simulink model "PID_Controller"  (R2017b)
settings: Solver=VariableStepAuto  StartTime=0.0  StopTime=10.0  RelTol=1e-3  EnableMultiTasking=on
values from neighbouring files (symbols this model uses):
  Fmatrix = [-1/sqrt(2) 0 1/sqrt(2) 1 ... (first row only)    [I_F_matrices.m]
  Imatrix = [1 0 0 1/2 ... (first row only)    [I_F_matrices.m]
libraries: dspmtrx3 x1, dspinverses x1
(part 2 of 5)

== matlab function PID_Controller/tau/Centrifugal and Coriolis Matrix/C_matrix ==
  data: in1 input; C output; in2 input
function C = Cmatrix(in1,in2)

C=zeros(6,6);
%CMATRIX
%    C = CMATRIX(IN1,IN2)

%    This function was generated by the Symbolic Math Toolbox version 7.0.
%    08-Aug-2017 18:04:25

dq1 = in2(1,:);
dq2 = in2(2,:);
dq3 = in2(3,:);
dq4 = in2(4,:);
dq5 = in2(5,:);
dq6 = in2(6,:);
q1 = in1(1,:);
q2 = in1(2,:);
q3 = in1(3,:);
q4 = in1(4,:);
q5 = in1(5,:);
q6 = in1(6,:);
t2 = cos(q1);
t3 = cos(q2);
t4 = sin(q1);
t5 = sin(q3);
t6 = cos(q3);
t7 = sin(q2);
t8 = t2.*(1.0./4.0);
t9 = t3.*t4.*(1.0./2.0);
t10 = t8+t9;
t11 = t4.*(1.0./4.0);
t19 = t2.*t3.*(1.0./2.0);
t12 = t11-t19;
t13 = t2.*t3.*t5;
t14 = t2.*t6.*t7;
t15 = t13+t14;
t16 = t3.*t4.*t5;
t17 = t4.*t6.*t7;
t18 = t16+t17;
t20 = t2.*t3.*t6;
t23 = t2.*t5.*t7;
t21 = t20-t23;
t22 = t3.*t4.*t6;
t24 = t3.*t6;
t26 = t5.*t7;
t25 = t24-t26;
t27 = t3.*t5;
t28 = t6.*t7;
t29 = t27+t28;
t30 = sin(q5);
t31 = sin(q4);
t32 = cos(q4);
t33 = cos(q5);
t34 = t8+t9+t16+t17;
t38 = t4.*t5.*t7;
t35 = t22-t38;
t36 = -t11+t13+t14+t19;
t37 = t2.*t31;
t39 = t18.*t33;
t40 = t4.*t31;
t44 = t21.*t32;
t41 = t40-t44;
t42 = t15.*t33;
t45 = t30.*t41;
t43 = t42-t45;
t46 = t32.*(t22-t38);
t47 = t37+t46;
t48 = t30.*t47;
t49 = t39+t48;
t50 = t21.*t33;
t58 = t15.*t30.*t32;
t51 = t50-t58;
t52 = t33.*t35;
t69 = t18.*t30.*t32;
t53 = t52-t69;
t54 = t2.*t7.*(1.0./2.0);
t55 = -t20+t23+t54;
t56 = t4.*t7.*(1.0./2.0);
t57 = -t22+t38+t56;
t59 = t7.*(1.0./2.0);
t60 = -t24+t26+t59;
t61 = t25.*t33;
t63 = t29.*t30.*t32;
t62 = t61-t63;
t64 = t3.*(1.0./2.0);
t65 = t27+t28+t64;
t66 = t29.*t33;
t67 = t25.*t30.*t32;
t68 = t66+t67;
t70 = t2.*t3.*(3.0./2.0e2);
t71 = t4.*t7.*(3.0./2.0e2);
t72 = t70+t71;
t73 = t2.*t3.*(7.0./2.0e2);
t74 = t4.*t7.*(7.0./2.0e2);
t75 = t73+t74;
t76 = t3.*t4.*(3.0./2.0e2);
t77 = t3.*t4.*(7.0./2.0e2);
t147 = t2.*t7.*(7.0./2.0e2);
t78 = t77-t147;
t79 = t34.*t43.*(1.0./2.0);
t80 = t34.*t51;
t81 = t34.*t43;
t82 = t34.*t51.*(1.0./2.0);
t166 = t36.*t49;
t83 = t81-t166;
t84 = t7.*t21.*(1.0./2.0);
t85 = t12.*t29;
t86 = t7.*t15.*(8.0./5.0);
t226 = t12.*t25.*(1.6e1./5.0);
t87 = t86-t226;
t88 = t7.*t15.*(1.0./2.0);
t230 = t12.*t25;
t89 = t88-t230;
t90 = t7.*t21.*(8.0./5.0);
t91 = t12.*t29.*(1.6e1./5.0);
t92 = t49.*t60.*(1.0./2.0);
t93 = t34.*t62.*(1.0./2.0);
t94 = t92+t93;
t95 = t34.*t68;
t96 = t49.*t60;
t97 = t34.*t62;
t98 = t96+t97;
t99 = t34.*t68.*(1.0./2.0);
t100 = t43.*t60.*(1.0./2.0);
t101 = t36.*t62.*(1.0./2.0);
t102 = t36.*t68;
t103 = t100+t101;
t104 = t43.*t60;
t105 = t36.*t62;
t106 = t36.*t68.*(1.0./2.0);
t107 = t104+t105;
t108 = t10.*t15;
t109 = t12.*t18;
t110 = t108+t109;
t111 = t10.*t21.*(1.6e1./5.0);
t112 = t12.*t35.*(1.6e1./5.0);
t113 = t10.*t21;
t114 = t10.*t15.*(1.6e1./5.0);
t115 = t12.*t18.*(1.6e1./5.0);
t116 = t114+t115;
t117 = t12.*t35;
t118 = t7.*t35.*(1.0./2.0);
t119 = t10.*t25.*(1.6e1./5.0);
t120 = t7.*t18.*(8.0./5.0);
t121 = t119+t120;
t122 = t10.*t25;
t123 = t7.*t18.*(1.0./2.0);
t124 = t122+t123;
t125 = t7.*t35.*(8.0./5.0);
t126 = t2.*t31.*(1.0./2.0e2);
t150 = t4.*t32.*(1.0./2.0e2);
t127 = t126-t150;
t128 = t2.*t32.*(3.0./1.0e3);
t129 = t4.*t31.*(3.0./1.0e3);
t130 = t128+t129;
t131 = t2.*t31.*(3.0./1.0e3);
t153 = t4.*t32.*(3.0./1.0e3);
t132 = t131-t153;
t133 = t2.*t32.*(1.0./2.0e2);
t134 = t4.*t31.*(1.0./2.0e2);
t135 = t133+t134;
t136 = t15.*t31.*(1.0./2.0e2);
t404 = t18.*t32.*(1.0./2.0e2);
t137 = t136-t404;
t138 = t15.*t32.*(3.0./1.0e3);
t139 = t18.*t31.*(3.0./1.0e3);
t140 = t138+t139;
t141 = t15.*t31.*(3.0./1.0e3);
t399 = t18.*t32.*(3.0./1.0e3);
t142 = t141-t399;
t143 = t15.*t32.*(1.0./2.0e2);
t144 = t18.*t31.*(1.0./2.0e2);
t145 = t143+t144;
t157 = t2.*t7.*(3.0./2.0e2);
t146 = t76-t157;
t148 = t3.*t78;
t149 = t7.*t72;
t151 = t32.*t127;
t179 = t31.*t130;
t152 = t151-t179;
t154 = t32.*t132;
t182 = t31.*t135;
t155 = t154-t182;
t156 = t3.*t72;
t158 = t7.*t146;
t159 = t32.*t135;
t160 = t31.*t132;
t161 = t159+t160;
t162 = t32.*t130;
t163 = t31.*t127;
t164 = t162+t163;
t194 = t36.*t49.*(1.0./2.0);
t165 = t79-t194;
t167 = t33.*t41;
t168 = t15.*t30;
t169 = t167+t168;
t170 = t18.*t30;
t172 = t33.*t47;
t171 = t170-t172;
t173 = t25.*t30;
t174 = t29.*t32.*t33;
t175 = t173+t174;
t176 = t4.*t32;
t177 = t21.*t31;
t178 = t176+t177;
t180 = t2.*t32;
t183 = t31.*t35;
t181 = t180-t183;
t184 = t32.*t181.*(1.0./2.0e2);
t185 = t31.*t178.*(1.0./2.0e2);
t186 = t184+t185;
t187 = t32.*t178.*(3.0./1.0e3);
t281 = t31.*t181.*(3.0./1.0e3);
t188 = t187-t281;
t189 = t32.*t181.*(3.0./1.0e3);
t190 = t31.*t178.*(3.0./1.0e3);
t191 = t189+t190;
t192 = t32.*t178.*(1.0./2.0e2);
t276 = t31.*t181.*(1.0./2.0e2);
t193 = t192-t276;
t195 = t34.*t169;
t534 = t36.*t171;
t196 = t195-t534;
t197 = t165.*t196.*(1.0./2.0);
t198 = t34.*t169.*(1.0./2.0);
t467 = t36.*t171.*(1.0./2.0);
t199 = t198-t467;
t200 = t83.*t199.*(1.0./2.0);
t201 = cos(q6);
t202 = sin(q6);
t203 = t60.*t171.*(1.0./2.0);
t204 = t34.*t175.*(1.0./2.0);
t205 = t203+t204;
t206 = t98.*t205.*(1.0./2.0);
t207 = t60.*t171;
t208 = t34.*t175;
t209 = t207+t208;
t210 = t94.*t209.*(1.0./2.0);
t211 = t2.*t201.*(2.0./1.25e2);
t212 = t4.*t202.*(2.0./1.25e2);
t213 = t211+t212;
t214 = t2.*t202.*(2.0./1.25e2);
t316 = t4.*t201.*(2.0./1.25e2);
t215 = t214-t316;
t216 = t60.*t169;
t217 = t36.*t175;
t218 = t216+t217;
t219 = t103.*t218.*(1.0./2.0);
t220 = t60.*t169.*(1.0./2.0);
t221 = t36.*t175.*(1.0./2.0);
t222 = t220+t221;
t223 = t107.*t222.*(1.0./2.0);
t224 = t2.*t7.*t18.*(1.0./2.0);
t225 = t2.*t7.*t18.*(8.0./5.0);
t227 = t3.*t15.*(1.0./2.0);
t353 = t2.*t7.*t25.*(1.0./2.0);
t228 = t84+t85+t227-t353;
t229 = t87.*t228.*(1.0./2.0);
t231 = t3.*t15.*(8.0./5.0);
t274 = t2.*t7.*t25.*(8.0./5.0);
t232 = t90+t91+t231-t274;
t233 = t89.*t232.*(1.0./2.0);
t234 = t49.*t55;
t354 = t36.*t53;
t355 = t43.*t57;
t235 = t80+t234-t354-t355;
t236 = t49.*t55.*(1.0./2.0);
t302 = t36.*t53.*(1.0./2.0);
t303 = t43.*t57.*(1.0./2.0);
t237 = t82+t236-t302-t303;
t238 = t51.*t60;
t239 = t55.*t62;
t240 = t51.*t60.*(1.0./2.0);
t241 = t55.*t62.*(1.0./2.0);
t242 = t53.*t60;
t243 = t57.*t62;
t244 = t53.*t60.*(1.0./2.0);
t245 = t57.*t62.*(1.0./2.0);
t246 = t3.*t146;
t247 = t7.*t75;
t248 = t3.*t18.*(1.0./2.0);
t358 = t10.*t29;
t359 = t4.*t7.*t25.*(1.0./2.0);
t360 = t118+t248-t358-t359;
t249 = t121.*t360.*(1.0./2.0);
t250 = t3.*t18.*(8.0./5.0);
t252 = t10.*t29.*(1.6e1./5.0);
t253 = t4.*t7.*t25.*(8.0./5.0);
t254 = t125+t250-t252-t253;
t251 = t124.*t254.*(1.0./2.0);
t331 = t43.*t65.*(1.0./2.0);
t255 = t106-t240+t241-t331;
t341 = t49.*t65.*(1.0./2.0);
t256 = t99-t244+t245-t341;
t257 = t30.*t60.*t178.*(1.0./2.0);
t443 = t29.*t30.*t31.*t36.*(1.0./2.0);
t258 = t257-t443;
t259 = t107.*t258.*(1.0./2.0);
t260 = t30.*t60.*t178;
t511 = t29.*t30.*t31.*t36;
t261 = t260-t511;
t262 = t103.*t261.*(1.0./2.0);
t273 = t29.*t31.*(1.09e2./1.0e3);
t263 = t59-t273;
t264 = t4.*t32.*(1.09e2./1.0e3);
t265 = t21.*t31.*(1.09e2./1.0e3);
t266 = -t11+t19+t264+t265;
t267 = t15.*t31.*(1.09e2./1.0e3);
t268 = t54+t267;
t269 = t31.*(t22-t38).*(1.09e2./1.0e3);
t315 = t2.*t32.*(1.09e2./1.0e3);
t270 = t8+t9+t269-t315;
t271 = t12.*(t22-t38).*(1.6e1./5.0);
t352 = t4.*t7.*t15.*(8.0./5.0);
t272 = t111+t225+t271-t352;
t275 = t35.*t43;
t277 = t32.*t193;
t278 = t31.*t191;
t279 = t277+t278;
t280 = t2.*t279.*(1.0./2.0);
t282 = t32.*t188;
t283 = t31.*t186;
t284 = t282+t283;
t285 = t32.*t186;
t429 = t31.*t188;
t286 = t285-t429;
t287 = t4.*t286.*(1.0./2.0);
t288 = t32.*t191;
t430 = t31.*t193;
t289 = t288-t430;
t290 = t151-t154-t179+t182;
t291 = t29.*t49;
t292 = t21.*t62;
t293 = t29.*t43;
t294 = t30.*t60.*t181.*(1.0./2.0);
t295 = t29.*t30.*t31.*t34.*(1.0./2.0);
t296 = t294+t295;
t297 = t30.*t60.*t181;
t298 = t29.*t30.*t31.*t34;
t299 = t297+t298;
t300 = t159+t160-t162-t163;
t301 = t4.*t300.*(1.0./2.0);
t304 = t30.*t36.*t181;
t305 = t30.*t34.*t178;
t306 = t304+t305;
t307 = t165.*t306.*(1.0./2.0);
t308 = t30.*t36.*t181.*(1.0./2.0);
t309 = t30.*t34.*t178.*(1.0./2.0);
t310 = t308+t309;
t311 = t83.*t310.*(1.0./2.0);
t312 = t18.*t31.*(1.09e2./1.0e3);
t313 = t56+t312;
t529 = t25.*t31.*(1.09e2./1.0e3);
t314 = t64-t529;
t317 = t202.*t213;
t322 = t201.*t215;
t318 = t317-t322;
t319 = t201.*t213;
t320 = t202.*t215;
t321 = t319+t320;
t323 = t51.*t318.*(1.0./2.0);
t324 = t33.*t35.*(1.1e1./5.0e2);
t412 = t18.*t30.*t32.*(1.1e1./5.0e2);
t325 = -t22+t38+t56+t324-t412;
t339 = t30.*t47.*(1.1e1./5.0e2);
t340 = t18.*t33.*(1.1e1./5.0e2);
t326 = t8+t9+t16+t17-t339-t340;
t327 = t30.*t41.*(1.1e1./5.0e2);
t334 = t15.*t33.*(1.1e1./5.0e2);
t328 = -t11+t13+t14+t19+t327-t334;
t329 = t29.*t30.*t32.*(1.1e1./5.0e2);
t338 = t25.*t33.*(1.1e1./5.0e2);
t330 = -t24+t26+t59+t329-t338;
t332 = t21.*t33.*(1.1e1./5.0e2);
t413 = t15.*t30.*t32.*(1.1e1./5.0e2);
t333 = -t20+t23+t54+t332-t413;
t335 = t29.*t33.*(1.1e1./5.0e2);
t336 = t25.*t30.*t32.*(1.1e1./5.0e2);
t337 = t27+t28+t64+t335+t336;
t342 = t246+t247;
t343 = t2.*t342.*(1.0./2.0);
t344 = t2.*t152.*(1.0./2.0);
t363 = t7.*t78;
t345 = t156-t363;
t346 = t4.*t345.*(1.0./2.0);
t361 = t3.*t75;
t347 = t158-t361;
t348 = t4.*t347.*(1.0./2.0);
t349 = t4.*t164.*(1.0./2.0);
t350 = t12.*(t22-t38);
t619 = t4.*t7.*t15.*(1.0./2.0);
t351 = t113+t224+t350-t619;
t598 = t43.*t65;
t356 = t102-t238+t239-t598;
t604 = t49.*t65;
t357 = t95-t242+t243-t604;
t362 = t7.*(t76-t157);
t364 = t25.*t43;
t444 = t15.*t62;
t365 = t364-t444;
t366 = t255.*t365.*(1.0./2.0);
t367 = t25.*t49;
t431 = t18.*t62;
t368 = t367-t431;
t369 = t256.*t368.*(1.0./2.0);
t370 = t35.*t43.*(1.0./2.0);
t371 = t84+t85;
t372 = t87.*t371.*(1.0./2.0);
t373 = t90+t91;
t374 = t89.*t373.*(1.0./2.0);
t375 = t35.*t62;
t376 = -t95+t242+t291+t375;
t377 = t94.*t376.*(1.0./2.0);
t378 = t29.*t49.*(1.0./2.0);
t379 = t35.*t62.*(1.0./2.0);
t380 = -t99+t244+t378+t379;
t381 = t98.*t380.*(1.0./2.0);
t382 = -t102+t238+t292+t293;
t383 = t103.*t382.*(1.0./2.0);
t384 = t21.*t62.*(1.0./2.0);
t385 = t29.*t43.*(1.0./2.0);
t386 = -t106+t240+t384+t385;
t387 = t107.*t386.*(1.0./2.0);
t388 = t18.*t51;
t437 = t21.*t49;
t438 = t15.*t53;
t389 = t275+t388-t437-t438;
t390 = t165.*t389.*(1.0./2.0);
t391 = t62.*(t22-t38);
t447 = t25.*t53;
t448 = t18.*t68;
t392 = t291+t391-t447-t448;
t393 = t94.*t392.*(1.0./2.0);
t449 = t25.*t51;
t450 = t15.*t68;
t394 = t292+t293-t449-t450;
t395 = t18.*t43;
t432 = t15.*t49;
t396 = t395-t432;
t397 = t237.*t396.*(1.0./2.0);
t398 = t32.*t145;
t400 = t31.*t142;
t401 = t398+t400;
t402 = t2.*t401.*(1.0./2.0);
t403 = t32.*t140;
t405 = t31.*t137;
t406 = t403+t405;
t407 = t32.*t137;
t455 = t31.*t140;
t408 = t407-t455;
t409 = t4.*t408.*(1.0./2.0);
t410 = t32.*t142;
t456 = t31.*t145;
t411 = t410-t456;
t414 = t22-t38-t324+t412;
t415 = t53.*t328;
t416 = t62.*t328;
t417 = t20-t23-t332+t413;
t418 = t27+t28+t335+t336;
t419 = t51.*t330;
t420 = t62.*t326;
t421 = t49.*t330;
t422 = t420+t421;
t423 = t43.*t326;
t504 = t49.*t328;
t424 = t423-t504;
t439 = t21.*t49.*(1.0./2.0);
t425 = t82-t302+t370-t439;
t426 = t43.*t330;
t427 = t416+t426;
t428 = t53.*t330;
t433 = t15.*t263;
t434 = t25.*t266;
t435 = t433+t434;
t436 = t21.*t263;
t440 = t21.*t270;
t441 = t111+t271;
t442 = t18.*t266;
t445 = t18.*t263;
t446 = t125-t252;
t451 = t35.*t263;
t452 = t15.*t31.*t152.*(1.0./2.0);
t453 = t18.*t31.*t321.*(1.0./2.0);
t454 = t18.*t31.*t164.*(1.0./2.0);
t457 = (t22-t38).*(t42-t45);
t458 = t388-t437-t438+t457;
t459 = (t22-t38).*(t42-t45).*(1.0./2.0);
t460 = t82-t302-t439+t459;
t461 = t110.*t441.*(1.0./2.0);
t462 = t113+t350;
t463 = t116.*t462.*(1.0./2.0);
t464 = t118-t358;
t465 = t121.*t464.*(1.0./2.0);
t466 = t124.*t446.*(1.0./2.0);
t468 = t80-t354-t437+t457;
t469 = t165.*t468.*(1.0./2.0);
t470 = t83.*t460.*(1.0./2.0);
t471 = t15.*t164.*(1.0./2.0);
t472 = t21.*t152.*(1.0./2.0);
t473 = t35.*t321.*(1.0./2.0);
t474 = t18.*t155.*(1.0./2.0);
t475 = t35.*t164.*(1.0./2.0);
t476 = t103.*t394.*(1.0./2.0);
t477 = t15.*t300.*(1.0./2.0);
t478 = t25.*t30.*t181;
t507 = t18.*t29.*t30.*t31;
t479 = t478-t507;
t480 = t18.*t290.*(1.0./2.0);
t481 = t15.*t30.*t181;
t482 = t18.*t30.*t178;
t483 = t481+t482;
t484 = t29.*t266;
t485 = t15.*t25.*t31.*(1.09e2./5.0e2);
t486 = -t436+t484+t485;
t487 = t87.*t486.*(1.0./2.0);
t488 = t458.*(t79-t194).*(1.0./2.0);
t489 = t460.*(t395-t432).*(1.0./2.0);
t527 = t35.*t266;
t490 = t440-t527;
t532 = t15.*t270;
t491 = t441.*(t442-t532).*(1.0./2.0);
t492 = t25.*t30.*t178;
t493 = t15.*t29.*t30.*t31;
t494 = t492+t493;
t495 = t494.*(t100+t101).*(1.0./2.0);
t496 = t258.*(t364-t444).*(1.0./2.0);
t497 = t25.*t270;
t498 = t445+t497;
t499 = (t100+t101).*(t292+t293-t449-t450).*(1.0./2.0);
t500 = t29.*t270;
t501 = t18.*t25.*t31.*(1.09e2./5.0e2);
t502 = -t451+t500+t501;
t503 = t121.*t502.*(1.0./2.0);
t505 = t4.*t31.*(1.09e2./1.0e3);
t927 = t21.*t32.*(1.09e2./1.0e3);
t506 = t505-t927;
t508 = t2.*t31.*(1.09e2./1.0e3);
t509 = t32.*(t22-t38).*(1.09e2./1.0e3);
t510 = t508+t509;
t512 = t2.*t290.*(1.0./2.0);
t513 = t98.*t296.*(1.0./2.0);
t514 = t94.*t299.*(1.0./2.0);
t515 = t222.*t365.*(1.0./2.0);
t516 = t15.*t175;
t536 = t25.*t169;
t517 = t516-t536;
t518 = t15.*t171;
t537 = t18.*t169;
t519 = t518-t537;
t520 = t165.*t519.*(1.0./2.0);
t521 = t18.*t175;
t538 = t25.*t171;
t522 = t521-t538;
t523 = t205.*t368.*(1.0./2.0);
t524 = t30.*t178.*t318.*(1.0./2.0);
t525 = t30.*t181.*t321.*(1.0./2.0);
t526 = t18.*t268;
t528 = t164.*t178.*(1.0./2.0);
t530 = t15.*t314;
t531 = t152.*t181.*(1.0./2.0);
t533 = t18.*t314;
t535 = t53.*t321.*(1.0./2.0);
t539 = t33.*t41.*(1.1e1./5.0e2);
t540 = t15.*t30.*(1.1e1./5.0e2);
t541 = t539+t540;
t542 = t25.*t30.*(1.1e1./5.0e2);
t543 = t29.*t32.*t33.*(1.1e1./5.0e2);
t544 = t542+t543;
t545 = t18.*t30.*(1.1e1./5.0e2);
t561 = t33.*t47.*(1.1e1./5.0e2);
t546 = t545-t561;
t547 = t197+t200+t206+t210+t219+t223;
t548 = t62.*t414;
t549 = t49.*t418;
t550 = t49.*t417;
t594 = t51.*t326;
t778 = t43.*t414;
t551 = t415+t550-t594-t778;
t552 = t62.*t417;
t553 = t43.*t418;
t554 = t386.*t427.*(1.0./2.0);
t555 = t380.*t422.*(1.0./2.0);
t595 = t68.*t328;
t556 = t419+t552+t553-t595;
t557 = t103.*t556.*(1.0./2.0);
t591 = t68.*t326;
t558 = t428+t548+t549-t591;
t559 = t94.*t558.*(1.0./2.0);
t560 = t49.*t541;
t562 = t169.*t326;
t563 = t560+t562-t171.*t328-t43.*t546;
t564 = t165.*t563.*(1.0./2.0);
t565 = t169.*t318.*(1.0./2.0);
t566 = t175.*t328;
t567 = t169.*t330;
t1010 = t43.*t544;
t1011 = t62.*t541;
t568 = t566+t567-t1010-t1011;
t569 = t175.*t326;
t570 = t171.*t330;
t571 = t569+t570-t49.*t544-t62.*t546;
t572 = t94.*t571.*(1.0./2.0);
t573 = t205.*t422.*(1.0./2.0);
t574 = t199.*t424.*(1.0./2.0);
t575 = t222.*t427.*(1.0./2.0);
t576 = t30.*t62.*t181.*(1.1e1./5.0e2);
t577 = t29.*t30.*t31.*t49.*(1.1e1./5.0e2);
t578 = t576+t577-t30.*t181.*t330-t29.*t30.*t31.*t326;
t579 = t94.*t578.*(1.0./2.0);
t580 = t30.*t49.*t178.*(1.1e1./5.0e2);
t581 = t30.*t181.*t328;
t582 = t30.*t178.*t326;
t583 = t30.*t43.*t181.*(1.1e1./5.0e2);
t584 = t580+t581+t582+t583;
t585 = t165.*t584.*(1.0./2.0);
t586 = t30.*t62.*t178.*(1.1e1./5.0e2);
t587 = t29.*t30.*t31.*t328;
t982 = t30.*t178.*t330;
t983 = t29.*t30.*t31.*t43.*(1.1e1./5.0e2);
t588 = t586+t587-t982-t983;
t589 = t258.*t427.*(1.0./2.0);
t590 = t310.*t424.*(1.0./2.0);
t592 = t49.*t337;
t593 = t43.*t325;
t596 = t43.*t337;
t597 = t237.*t424.*(1.0./2.0);
t599 = t51.*t201.*(2.0./1.25e2);
t600 = t51.*t202.*(2.0./1.25e2);
t605 = t53.*t201.*(2.0./1.25e2);
t601 = t600-t605;
t602 = t53.*t202.*(2.0./1.25e2);
t603 = t599+t602;
t606 = t201.*t601;
t729 = t202.*t603;
t607 = t606-t729;
t608 = t2.*t607.*(1.0./2.0);
t609 = t202.*t601;
t610 = t201.*t603;
t611 = t609+t610;
t612 = t4.*t611.*(1.0./2.0);
t613 = t31.^2;
t614 = t18.*t613.*(1.0./2.0e2);
t615 = t15.*t31.*t32.*(1.0./2.0e2);
t616 = t614+t615;
t617 = t15.*t613.*(3.0./1.0e3);
t669 = t18.*t31.*t32.*(3.0./1.0e3);
t618 = t617-t669;
t620 = t15.*t31.*t201.*(2.0./1.25e2);
t621 = t18.*t31.*t202.*(2.0./1.25e2);
t622 = t620+t621;
t623 = t15.*t31.*t202.*(2.0./1.25e2);
t673 = t18.*t31.*t201.*(2.0./1.25e2);
t624 = t623-t673;
t625 = t148+t149;
t730 = t2.*t155.*(1.0./2.0);
t731 = t4.*t161.*(1.0./2.0);
t732 = t2.*t625.*(1.0./2.0);
t626 = t343+t344+t346+t348+t349-t730-t731-t732;
t627 = t116.*t351.*(1.0./2.0);
t628 = t110.*t272.*(1.0./2.0);
t629 = t83.*t237.*(1.0./2.0);
t630 = t3.*(t77-t147);
t631 = t149-t246-t247+t630;
t632 = t156-t361+t362-t363;
t633 = t25.*t43.*(1.0./2.0);
t662 = t15.*t62.*(1.0./2.0);
t634 = t633-t662;
t635 = t356.*t634.*(1.0./2.0);
t636 = t25.*t49.*(1.0./2.0);
t664 = t18.*t62.*(1.0./2.0);
t637 = t636-t664;
t638 = t357.*t637.*(1.0./2.0);
t639 = t15.*t161.*(1.0./2.0);
t640 = t15.*t53.*(1.0./2.0);
t641 = t18.*t152.*(1.0./2.0);
t691 = t25.*t53.*(1.0./2.0);
t692 = t18.*t68.*(1.0./2.0);
t642 = t378+t379-t691-t692;
t643 = t98.*t642.*(1.0./2.0);
t693 = t25.*t51.*(1.0./2.0);
t694 = t15.*t68.*(1.0./2.0);
t644 = t384+t385-t693-t694;
t645 = t107.*t644.*(1.0./2.0);
t646 = t18.*t43.*(1.0./2.0);
t695 = t15.*t49.*(1.0./2.0);
t647 = t646-t695;
t648 = t235.*t647.*(1.0./2.0);
t649 = t21.*t201.*(2.0./1.25e2);
t650 = t21.*t202.*(2.0./1.25e2);
t713 = t35.*t201.*(2.0./1.25e2);
t651 = t650-t713;
t652 = t21.*t32.*(1.0./2.0e2);
t653 = t21.*t31.*(3.0./1.0e3);
t717 = t32.*t35.*(3.0./1.0e3);
t654 = t653-t717;
t655 = t18.*t263.*(1.6e1./5.0);
t656 = t25.*t270.*(1.6e1./5.0);
t657 = t655+t656;
t936 = t15.*t313;
t658 = t440+t526-t527-t936;
t659 = t18.*t268.*(1.6e1./5.0);
t660 = t21.*t270.*(1.6e1./5.0);
t938 = t15.*t313.*(1.6e1./5.0);
t661 = t659+t660-t938-t35.*t266.*(1.6e1./5.0);
t663 = t255.*(t364-t444).*(1.0./2.0);
t941 = t25.*t268;
t665 = t436-t484+t530-t941;
t666 = t21.*t263.*(1.6e1./5.0);
t667 = t15.*t314.*(1.6e1./5.0);
t942 = t29.*t266.*(1.6e1./5.0);
t943 = t25.*t268.*(1.6e1./5.0);
t668 = t666+t667-t942-t943;
t670 = t31.*t616;
t867 = t32.*t618;
t671 = t670-t867;
t672 = t2.*t671.*(1.0./2.0);
t674 = t202.*t622;
t868 = t201.*t624;
t675 = t674-t868;
t676 = t2.*t675.*(1.0./2.0);
t677 = t32.*t616;
t678 = t31.*t618;
t679 = t677+t678;
t680 = t18.*t266.*(1.6e1./5.0);
t681 = t680-t15.*t270.*(1.6e1./5.0);
t682 = t351.*t681.*(1.0./2.0);
t683 = t272.*(t442-t532).*(1.0./2.0);
t684 = t201.*t622;
t685 = t202.*t624;
t686 = t684+t685;
t687 = t15.*t263.*(1.6e1./5.0);
t688 = t25.*t266.*(1.6e1./5.0);
t689 = t687+t688;
t712 = t18.*t51.*(1.0./2.0);
t690 = (t81-t166).*(t439-t459+t640-t712).*(1.0./2.0);
t696 = t237.*(t395-t432).*(1.0./2.0);
t932 = t25.*t313;
t697 = t451-t500+t533-t932;
t698 = t18.*t314.*(1.6e1./5.0);
t699 = t35.*t263.*(1.6e1./5.0);
t700 = t468.*(t79-t194).*(1.0./2.0);
t701 = t460.*(t81-t166).*(1.0./2.0);
t702 = t94.*(-t95+t242+t291+t375).*(1.0./2.0);
t703 = t98.*(-t99+t244+t378+t379).*(1.0./2.0);
t704 = t29.*(t42-t45);
t705 = -t102+t238+t292+t704;
t706 = t705.*(t100+t101).*(1.0./2.0);
t707 = t29.*(t42-t45).*(1.0./2.0);
t708 = -t106+t240+t384+t707;
t709 = t708.*(t104+t105).*(1.0./2.0);
t710 = t121.*(t118-t358).*(1.0./2.0);
t711 = t124.*(t125-t252).*(1.0./2.0);
t714 = t201.*t651;
t715 = t202.*(t22-t38).*(2.0./1.25e2);
t716 = t649+t715;
t718 = t32.*t654;
t719 = t31.*(t22-t38).*(1.0./2.0e2);
t720 = t652+t719;
t721 = t201.*t716;
t722 = t202.*t651;
t723 = t721+t722;
t724 = t4.*t723.*(1.0./2.0);
t725 = t32.*t720;
t726 = t31.*t654;
t727 = t725+t726;
t728 = t4.*t727.*(1.0./2.0);
t733 = t428-t591+t592-t62.*t325;
t734 = t94.*t733.*(1.0./2.0);
t735 = t49.*t337.*(1.0./2.0);
t736 = t53.*t330.*(1.0./2.0);
t737 = t43.*t325.*(1.0./2.0);
t738 = t53.*t328.*(1.0./2.0);
t757 = t49.*t333.*(1.0./2.0);
t758 = t51.*t326.*(1.0./2.0);
t739 = t737+t738-t757-t758;
t740 = t62.*t328.*(1.0./2.0);
t741 = t43.*t330.*(1.0./2.0);
t742 = t740+t741;
t1034 = t62.*t333;
t743 = t419-t595+t596-t1034;
t744 = t103.*t743.*(1.0./2.0);
t745 = t43.*t337.*(1.0./2.0);
t746 = t51.*t330.*(1.0./2.0);
t747 = t43.*t326.*(1.0./2.0);
t759 = t49.*t328.*(1.0./2.0);
t777 = t747-t759;
t748 = t235.*t777.*(1.0./2.0);
t749 = t62.*t326.*(1.0./2.0);
t750 = t49.*t330.*(1.0./2.0);
t751 = t749+t750;
t752 = t235.*(t79-t194).*(1.0./2.0);
t753 = t237.*(t81-t166).*(1.0./2.0);
t754 = t4.*t632.*(1.0./2.0);
t755 = t2.^2;
t756 = t4.^2;
t760 = t202.*(t52-t69).*(2.0./1.25e2);
t761 = t599+t760;
t762 = t201.*t761;
t763 = t609+t762;
t984 = t62.*t333.*(1.0./2.0);
t985 = t68.*t328.*(1.0./2.0);
t764 = t745+t746-t984-t985;
t765 = t330.*(t42-t45);
t766 = t416+t765;
t767 = t424.*t460.*(1.0./2.0);
t768 = t43.*t202.*(2.0./1.25e2);
t769 = -t22+t38;
t770 = t43.*t201.*(2.0./1.25e2);
t774 = t32.*t769;
t771 = t37-t774;
t772 = t30.*t771;
t773 = t39+t772;
t775 = t33.*t769;
t776 = t69+t775;
t779 = t15.*t202.*(2.0./1.25e2);
t912 = t18.*t201.*(2.0./1.25e2);
t780 = t779-t912;
t781 = t15.*t201.*(2.0./1.25e2);
t782 = t18.*t202.*(2.0./1.25e2);
t783 = t781+t782;
t784 = t201.*t769.*(2.0./1.25e2);
t785 = t650+t784;
t873 = t202.*t769.*(2.0./1.25e2);
t786 = t649-t873;
t787 = t32.*t769.*(3.0./1.0e3);
t788 = t653+t787;
t875 = t31.*t769.*(1.0./2.0e2);
t789 = t652-t875;
t790 = t21.*t152;
t791 = t62.*t769;
t806 = t29.*t773;
t852 = t25.*t776;
t792 = t448+t791-t806-t852;
t793 = t62.*t769.*(1.0./2.0);
t829 = t25.*t773;
t794 = t431-t829;
t795 = (t100+t101).*(t292+t293-t449-t450);
t796 = t15.*t776;
t799 = t43.*t769;
t800 = t21.*t773;
t797 = t388+t796-t799-t800;
t825 = t15.*t773;
t798 = t395-t825;
t826 = t36.*t773.*(1.0./2.0);
t801 = t79-t826;
t802 = t36.*t776.*(1.0./2.0);
t833 = t43.*t769.*(1.0./2.0);
t834 = t21.*t773.*(1.0./2.0);
t803 = t82+t802-t833-t834;
t804 = t60.*t773.*(1.0./2.0);
t805 = t93+t804;
t807 = t60.*t776.*(1.0./2.0);
t841 = t29.*t773.*(1.0./2.0);
t808 = t99+t793+t807-t841;
t809 = t201.*t776.*(2.0./1.25e2);
t810 = t600+t809;
t962 = t202.*t776.*(2.0./1.25e2);
t811 = t599-t962;
t812 = t202.*t773.*(2.0./1.25e2);
t813 = t770+t812;
t815 = t201.*t773.*(2.0./1.25e2);
t814 = t768-t815;
t816 = t201.*t814;
t977 = t202.*t813;
t817 = t816-t977;
t818 = t769.*t817.*(1.0./2.0);
t819 = t321.*t776.*(1.0./2.0);
t820 = t25.*t33.*(1.0./1.25e2);
t976 = t29.*t30.*t32.*(1.0./1.25e2);
t821 = t820-t976;
t822 = t29.*t33.*(1.0./1.25e2);
t823 = t25.*t30.*t32.*(1.0./1.25e2);
t824 = t822+t823;
t828 = t33.*t771;
t827 = t170-t828;
t830 = t36.*t776;
t831 = t80-t799-t800+t830;
t832 = t801.*t831.*(1.0./2.0);
t956 = t36.*t773;
t835 = t81-t956;
t836 = t803.*t835.*(1.0./2.0);
t837 = t60.*t776;
t838 = t95+t791-t806+t837;
t839 = t60.*t773;
t840 = t97+t839;
t842 = t103.*t705.*(1.0./2.0);
t843 = t107.*t708.*(1.0./2.0);
t863 = t12.*t769.*(1.6e1./5.0);
t844 = t111-t863;
t845 = t110.*t844.*(1.0./2.0);
t1097 = t12.*t769;
t846 = t113-t1097;
t847 = t116.*t846.*(1.0./2.0);
t848 = t7.*t769.*(1.0./2.0);
t849 = t358+t848;
t850 = t7.*t769.*(8.0./5.0);
t851 = t252+t850;
t853 = t31.*t769;
t854 = t180+t853;
t855 = t201.*t854.*(2.0./1.25e2);
t856 = t178.*t202.*(2.0./1.25e2);
t857 = t855+t856;
t858 = t178.*t201.*(2.0./1.25e2);
t946 = t202.*t854.*(2.0./1.25e2);
t859 = t858-t946;
t860 = t32.*t854.*(3.0./1.0e3);
t861 = t190+t860;
t948 = t31.*t854.*(1.0./2.0e2);
t862 = t192-t948;
t865 = t31.*t769.*(1.09e2./1.0e3);
t864 = t8+t9-t315-t865;
t866 = t792.*t805.*(1.0./2.0);
t903 = t15.*t773.*(1.0./2.0);
t869 = t646-t903;
t870 = t797.*t869.*(1.0./2.0);
t871 = t15.*t776.*(1.0./2.0);
t872 = t201.*t785;
t1029 = t202.*t786;
t874 = t872-t1029;
t876 = t31.*t789;
t1115 = t32.*t788;
t877 = t876-t1115;
t933 = t25.*t773.*(1.0./2.0);
t1045 = t664-t933;
t878 = t1045.*(t448+t791-t806-t852).*(1.0./2.0);
t934 = t25.*t776.*(1.0./2.0);
t1044 = t692+t793-t841-t934;
t879 = t1044.*(t431-t829).*(1.0./2.0);
t880 = (t633-t662).*(t292+t293-t449-t450).*(1.0./2.0);
t881 = (t364-t444).*(t384+t385-t693-t694).*(1.0./2.0);
t882 = t30.*t60.*t854.*(1.0./2.0);
t883 = t295+t882;
t884 = t883.*(t431-t829).*(1.0./2.0);
t935 = t25.*t30.*t854;
t1209 = t507-t935;
t885 = t805.*t1209.*(1.0./2.0);
t886 = t30.*t36.*t854.*(1.0./2.0);
t887 = t309+t886;
t888 = t15.*t30.*t854;
t889 = t482+t888;
t890 = t797.*(t79-t826).*(1.0./2.0);
t891 = t803.*(t395-t825).*(1.0./2.0);
t892 = t21.*t864;
t893 = t266.*t769;
t894 = t892+t893;
t937 = t15.*t864;
t997 = t442-t937;
t895 = t844.*t997.*(1.0./2.0);
t896 = t25.*t864;
t897 = t445+t896;
t898 = t851.*t897.*(1.0./2.0);
t899 = t263.*t769;
t900 = t29.*t864;
t901 = t501+t899+t900;
t902 = t121.*t901.*(1.0./2.0);
t904 = t712-t833-t834+t871;
t905 = t201.*t786;
t906 = t202.*t785;
t907 = t905+t906;
t908 = t32.*t789;
t909 = t31.*t788;
t910 = t908+t909;
t911 = t201.*t783;
t913 = t202.*t780;
t914 = t911+t913;
t915 = t201.*t780;
t1030 = t202.*t783;
t916 = t915-t1030;
t917 = t3.*t5.*(1.0./1.25e2);
t918 = t6.*t7.*(1.0./1.25e2);
t919 = t917+t918;
t920 = t3.*t6.*(1.0./1.25e2);
t1031 = t5.*t7.*(1.0./1.25e2);
t921 = t920-t1031;
t922 = t3.*t5.*(1.0./2.5e2);
t923 = t6.*t7.*(1.0./2.5e2);
t924 = t922+t923;
t925 = t3.*t6.*(1.0./2.5e2);
t1137 = t5.*t7.*(1.0./2.5e2);
t926 = t925-t1137;
t928 = t18.*t506;
t929 = t25.*t506;
t930 = t15.*t29.*t32.*(1.09e2./1.0e3);
t931 = t929+t930;
t939 = t41.*t318;
t1366 = t32.*t769.*(1.09e2./1.0e3);
t940 = t508-t1366;
t944 = t178.*t300;
t945 = t201.*t857;
t1019 = t202.*t859;
t947 = t945-t1019;
t949 = t31.*t862;
t950 = t201.*t859;
t951 = t202.*t857;
t952 = t950+t951;
t953 = t32.*t862;
t954 = t31.*t861;
t955 = t953+t954;
t957 = t103.*t517.*(1.0./2.0);
t1008 = t36.*t827.*(1.0./2.0);
t958 = t198-t1008;
t959 = t798.*t958.*(1.0./2.0);
t1020 = t15.*t827;
t960 = t537-t1020;
t961 = t801.*t960.*(1.0./2.0);
t963 = t201.*t811;
t964 = t202.*t810;
t965 = t963+t964;
t966 = t201.*t810;
t990 = t202.*t811;
t967 = t966-t990;
t1021 = t25.*t827;
t968 = t521-t1021;
t969 = t805.*t968.*(1.0./2.0);
t970 = t60.*t827.*(1.0./2.0);
t971 = t204+t970;
t972 = t794.*t971.*(1.0./2.0);
t973 = t201.*t813;
t974 = t202.*t814;
t975 = t973+t974;
t978 = t33.*t769.*(1.1e1./5.0e2);
t979 = t22-t38-t56+t412+t978;
t981 = t30.*t771.*(1.1e1./5.0e2);
t980 = t8+t9+t16+t17-t340-t981;
t986 = t178.*t965.*(1.0./2.0);
t987 = t62.*t979.*(1.0./2.0);
t988 = t337.*t773.*(1.0./2.0);
t1060 = t68.*t980.*(1.0./2.0);
t1061 = t330.*t776.*(1.0./2.0);
t989 = t987+t988-t1060-t1061;
t991 = t854.*t967.*(1.0./2.0);
t992 = t30.*t321.*t854.*(1.0./2.0);
t993 = t18.*t31.*t817.*(1.0./2.0);
t994 = t29.*t31.*t824.*(1.0./2.0);
t995 = t526+t892+t893-t936;
t1096 = t65.*t773.*(1.0./2.0);
t996 = t99+t245+t807-t1096;
t998 = t30.*t60.*t854;
t999 = t298+t998;
t1000 = t55.*t773.*(1.0./2.0);
t1001 = t82-t303+t802+t1000;
t1002 = t30.*t36.*t854;
t1003 = t305+t1002;
t1004 = t801.*t1003.*(1.0./2.0);
t1005 = t835.*t887.*(1.0./2.0);
t1006 = -t533+t899+t900+t932;
t1007 = t794.*t996.*(1.0./2.0);
t1009 = t773.*t967.*(1.0./2.0);
t1012 = t568.*(t100+t101).*(1.0./2.0);
t1013 = t62.*t980;
t1014 = t330.*t773;
t1015 = t1013+t1014;
t1016 = t43.*t980;
t1017 = t68.*t821.*(1.0./2.0);
t1018 = t62.*t824.*(1.0./2.0);
t1113 = t36.*t827;
t1022 = t195-t1113;
t1023 = t801.*t1022.*(1.0./2.0);
t1024 = t835.*t958.*(1.0./2.0);
t1025 = t840.*t971.*(1.0./2.0);
t1026 = t60.*t827;
t1027 = t208+t1026;
t1028 = t805.*t1027.*(1.0./2.0);
t1040 = t328.*t773;
t1032 = t1016-t1040;
t1033 = t51.*t914.*(1.0./2.0);
t1035 = t22-t38+t412+t978;
t1036 = t328.*t776;
t1037 = t51.*t980;
t1038 = t776.*t916.*(1.0./2.0);
t1039 = t708.*t766.*(1.0./2.0);
t1041 = t68.*t980;
t1042 = t330.*t776;
t1043 = t43.*t907.*(1.0./2.0);
t1046 = t43.*t980.*(1.0./2.0);
t1047 = t333.*t773;
t1098 = t328.*t773.*(1.0./2.0);
t1048 = t1046-t1098;
t1049 = t43.*t979;
t1050 = t1036+t1037+t1047+t1049;
t1051 = t333.*t773.*(1.0./2.0);
t1052 = t328.*t776.*(1.0./2.0);
t1053 = t51.*t980.*(1.0./2.0);
t1054 = t43.*t979.*(1.0./2.0);
t1055 = t1051+t1052+t1053+t1054;
t1056 = t62.*t980.*(1.0./2.0);
t1057 = t330.*t773.*(1.0./2.0);
t1058 = t1056+t1057;
t1089 = t62.*t979;
t1090 = t337.*t773;
t1059 = t1041+t1042-t1089-t1090;
t1062 = t541.*t773;
t1070 = t33.*t771.*(1.1e1./5.0e2);
t1063 = t545-t1070;
t1064 = t169.*t980;
t1253 = t43.*t1063;
t1254 = t328.*t827;
t1065 = t1062+t1064-t1253-t1254;
t1066 = t1065.*(t79-t826).*(1.0./2.0);
t1067 = t169.*(t317-t322).*(1.0./2.0);
t1068 = t51.*t975.*(1.0./2.0);
t1069 = t544.*t773;
t1071 = t62.*t1063;
t1255 = t175.*t980;
t1256 = t330.*t827;
t1072 = t1069+t1071-t1255-t1256;
t1073 = t776.*t817.*(1.0./2.0);
t1074 = t1015.*(t204+t970).*(1.0./2.0);
t1075 = t43.*t965.*(1.0./2.0);
t1076 = t222.*t766.*(1.0./2.0);
t1077 = t1015.*t1044.*(1.0./2.0);
t1078 = t30.*t62.*t854.*(1.1e1./5.0e2);
t1079 = t29.*t30.*t31.*t773.*(1.1e1./5.0e2);
t1237 = t30.*t330.*t854;
t1238 = t29.*t30.*t31.*t980;
t1080 = t1078+t1079-t1237-t1238;
t1081 = t805.*t1080.*(1.0./2.0);
t1082 = t30.*t178.*t773.*(1.1e1./5.0e2);
t1083 = t30.*t328.*t854;
t1084 = t30.*t178.*t980;
t1085 = t634.*t743.*(1.0./2.0);
t1086 = t258.*t766.*(1.0./2.0);
t1087 = t43.*t686.*(1.0./2.0);
t1088 = t675.*t773.*(1.0./2.0);
t1091 = t1045.*t1059.*(1.0./2.0);
t1092 = t25.*t31.*t62.*(1.0./2.5e2);
t1093 = t979.*(t42-t45);
t1094 = t1036+t1037+t1047+t1093;
t1095 = t255.*t766.*(1.0./2.0);
t1099 = t4.*t679.*(1.0./2.0);
t1100 = t4.*t686.*(1.0./2.0);
t1101 = t21.*t864.*(1.6e1./5.0);
t1102 = t266.*t769.*(1.6e1./5.0);
t1151 = t15.*t864.*(1.6e1./5.0);
t1103 = t680-t1151;
t1104 = t25.*t864.*(1.6e1./5.0);
t1105 = t655+t1104;
t1106 = t263.*t769.*(1.6e1./5.0);
t1107 = t29.*t864.*(1.6e1./5.0);
t1108 = t178.*t408.*(1.0./2.0);
t1109 = t15.*t411.*(1.0./2.0);
t1110 = t18.*t401.*(1.0./2.0);
t1111 = t2.*t967.*(1.0./2.0);
t1112 = t4.*t965.*(1.0./2.0);
t1114 = t835.*t904.*(1.0./2.0);
t1116 = t15.*t175.*(1.0./2.0);
t1200 = t25.*t169.*(1.0./2.0);
t1117 = t1116-t1200;
t1118 = t18.*t169.*(1.0./2.0);
t1197 = t15.*t827.*(1.0./2.0);
t1119 = t1118-t1197;
t1120 = t18.*t175.*(1.0./2.0);
t1198 = t25.*t827.*(1.0./2.0);
t1121 = t1120-t1198;
t1122 = t840.*t1121.*(1.0./2.0);
t1123 = t107.*t1117.*(1.0./2.0);
t1124 = t1027.*t1045.*(1.0./2.0);
t1125 = t835.*t1119.*(1.0./2.0);
t1126 = t869.*t1022.*(1.0./2.0);
t1185 = t65.*t773;
t1127 = t95+t243+t837-t1185;
t1128 = t55.*t773;
t1129 = t80-t355+t830+t1128;
t1130 = t21.*t914.*(1.0./2.0);
t1131 = t15.*t907.*(1.0./2.0);
t1132 = t21.*t401.*(1.0./2.0);
t1133 = t15.*t910.*(1.0./2.0);
t1134 = t769.*t916.*(1.0./2.0);
t1135 = t411.*t769.*(1.0./2.0);
t1136 = t18.*t877.*(1.0./2.0);
t1138 = t854.*t874.*(1.0./2.0);
t1139 = t398+t400-t403-t405;
t1140 = t407-t410-t455+t456;
t1141 = t25.*t30.*t854.*(1.0./2.0);
t1208 = t18.*t29.*t30.*t31.*(1.0./2.0);
t1142 = t1141-t1208;
t1143 = t840.*t1142.*(1.0./2.0);
t1144 = t15.*t30.*t854.*(1.0./2.0);
t1145 = t18.*t30.*t178.*(1.0./2.0);
t1146 = t1144+t1145;
t1147 = t15.*t25.*t31.*(4.36e2./6.25e2);
t1148 = -t666+t942+t1147;
t1149 = t89.*t1148.*(1.0./2.0);
t1150 = t1101+t1102;
t1152 = t25.*t30.*t178.*(1.0./2.0);
t1153 = t15.*t29.*t30.*t31.*(1.0./2.0);
t1154 = t1152+t1153;
t1155 = t849.*t1105.*(1.0./2.0);
t1156 = t840.*t1044.*(1.0./2.0);
t1157 = t18.*t25.*t31.*(4.36e2./6.25e2);
t1158 = t1106+t1107+t1157;
t1159 = t124.*t1158.*(1.0./2.0);
t1160 = t798.*t904.*(1.0./2.0);
t1161 = t178.*t907.*(1.0./2.0);
t1162 = t178.*t910.*(1.0./2.0);
t1163 = t18.*t31.*t916.*(1.0./2.0);
t1164 = t18.*t31.*t411.*(1.0./2.0);
t1165 = t29.*t31.*t919.*(1.0./2.0);
t1166 = t29.*t31.*t924.*(1.0./2.0);
t1167 = t835.*t1146.*(1.0./2.0);
t1168 = t831.*t869.*(1.0./2.0);
t1169 = t869.*t1003.*(1.0./2.0);
t1170 = t846.*t1103.*(1.0./2.0);
t1221 = t62.*t1035.*(1.0./2.0);
t1222 = t418.*t773.*(1.0./2.0);
t1171 = t1060+t1061-t1221-t1222;
t1172 = t773.*t874.*(1.0./2.0);
t1173 = t1035.*(t42-t45).*(1.0./2.0);
t1225 = t417.*t773.*(1.0./2.0);
t1174 = t1052+t1053+t1173-t1225;
t1175 = t1174.*(t81-t956).*(1.0./2.0);
t1176 = t330.*(t42-t45).*(1.0./2.0);
t1177 = t740+t1176;
t1178 = t705.*t1177.*(1.0./2.0);
t1179 = t62.*t417.*(1.0./2.0);
t1180 = t43.*t418.*(1.0./2.0);
t1219 = t746-t985+t1179+t1180;
t1181 = t1219.*(t104+t105).*(1.0./2.0);
t1182 = t831.*(t1046-t1098).*(1.0./2.0);
t1183 = t68.*t921.*(1.0./2.0);
t1184 = t62.*t919.*(1.0./2.0);
t1186 = t2.*t874.*(1.0./2.0);
t1187 = t4.*t907.*(1.0./2.0);
t1188 = t4.*t910.*(1.0./2.0);
t1189 = t1045.*t1127.*(1.0./2.0);
t1194 = t2.*t877.*(1.0./2.0);
t1291 = t869.*t1129.*(1.0./2.0);
t1190 = t372+t374+t402+t409-t635-t645+t706+t709+t832+t836+t845+t847-t1114+t1156+t1186+t1187+t1188+t1189-t1194-t1291-t2.*t406.*(1.0./2.0)-t4.*t411.*(1.0./2.0)-t121.*t849.*(1.0./2.0)-t124.*t851.*(1.0./2.0)-t805.*t838.*(1.0./2.0)-t808.*t840.*(1.0./2.0);
t1191 = t21.*t318.*(1.0./2.0);
t1192 = t321.*t769.*(1.0./2.0);
t1193 = t164.*t769.*(1.0./2.0);
t1195 = t907.*(t42-t45).*(1.0./2.0);
t1196 = t15.*t965.*(1.0./2.0);
t1199 = t21.*t975.*(1.0./2.0);
t1201 = t21.*t952.*(1.0./2.0);
t1202 = t21.*t955.*(1.0./2.0);
t1203 = t769.*t947.*(1.0./2.0);
t1234 = t32.*t861;
t1204 = t949-t1234;
t1205 = t29.^2;
t1206 = t31.*t1205.*(3.0./5.0e2);
t1207 = t25.^2;
t1210 = t634.*t705.*(1.0./2.0);
t1211 = t838.*t1045.*(1.0./2.0);
t1212 = t792.*t1045.*(1.0./2.0);
t1213 = t794.*t1044.*(1.0./2.0);
t1214 = t18.*t874.*(1.0./2.0);
t1215 = t29.*t921.*(1.0./2.0);
t1216 = t25.*t919.*(1.0./2.0);
t1217 = t29.*t926.*(1.0./2.0);
t1218 = t25.*t924.*(1.0./2.0);
t1220 = t1015.*(t692+t793-t841-t934).*(1.0./2.0);
t1223 = t43.*t1035;
t1263 = t417.*t773;
t1224 = t1036+t1037+t1223-t1263;
t1226 = t797.*t1048.*(1.0./2.0);
t1261 = t62.*t1035;
t1262 = t418.*t773;
t1227 = t1041+t1042-t1261-t1262;
t1228 = t869.*t960.*(1.0./2.0);
t1229 = t798.*t1119.*(1.0./2.0);
t1230 = t968.*t1045.*(1.0./2.0);
t1231 = t794.*t1121.*(1.0./2.0);
t1232 = t178.*t679.*(1.0./2.0);
t1233 = t178.*t686.*(1.0./2.0);
t1235 = t15.*t31.*t952.*(1.0./2.0);
t1236 = t15.*t31.*t955.*(1.0./2.0);
t1239 = t30.*t854.*(t42-t45).*(1.1e1./5.0e2);
t1240 = t1082+t1083+t1084+t1239;
t1241 = t25.*t31.*t821.*(1.0./2.0);
t1242 = t30.*t178.*t914.*(1.0./2.0);
t1243 = t30.*t854.*t916.*(1.0./2.0);
t1244 = t494.*t634.*(1.0./2.0);
t1245 = t365.*t1154.*(1.0./2.0);
t1246 = t15.*t1140.*(1.0./2.0);
t1247 = t794.*t1142.*(1.0./2.0);
t1248 = t869.*t889.*(1.0./2.0);
t1249 = t798.*t1146.*(1.0./2.0);
t1250 = t401.*t854.*(1.0./2.0);
t1251 = (t664-t933).*(t448+t791-t806-t852).*(1.0./2.0);
t1252 = (t431-t829).*(t692+t793-t841-t934).*(1.0./2.0);
t1257 = t776.*t947.*(1.0./2.0);
t1258 = t51.*t952.*(1.0./2.0);
t1259 = t29.*t31.*t68.*(1.0./2.5e2);
t1260 = t29.*t30.*t31.*t921.*(1.0./2.0);
t1264 = t904.*t1032.*(1.0./2.0);
t1265 = t1015.*t1142.*(1.0./2.0);
t1266 = t1045.*t1080.*(1.0./2.0);
t1267 = t869.*t1240.*(1.0./2.0);
t1268 = t588.*t634.*(1.0./2.0);
t1269 = t1035.*(t42-t45);
t1270 = t1036+t1037-t1263+t1269;
t1271 = t1032.*t1146.*(1.0./2.0);
t1272 = t644.*t766.*(1.0./2.0);
t1273 = t916.*(t170-t828).*(1.0./2.0);
t1274 = t1015.*t1121.*(1.0./2.0);
t1275 = t1119.*(t1016-t1040).*(1.0./2.0);
t1276 = t766.*t1117.*(1.0./2.0);
t1277 = t1065.*(t646-t903).*(1.0./2.0);
t1493 = t169.*t914.*(1.0./2.0);
t1496 = t175.*t921.*(1.0./2.0);
t1504 = t568.*t634.*(1.0./2.0);
t1278 = t1009+t1017+t1018-t1068-t1073-t1075+t1273+t1274+t1275+t1276+t1277-t1493-t1496-t1504-t1045.*t1072.*(1.0./2.0);
t1279 = (t633-t662).*(t419-t595+t596-t1034).*(1.0./2.0);
t1280 = t1270.*(t79-t826).*(1.0./2.0);
t1281 = t51.*(t317-t322).*(1.0./2.0);
t1282 = (t100+t101).*(t419+t552+t553-t595).*(1.0./2.0);
t1283 = t803.*(t1016-t1040).*(1.0./2.0);
t1284 = t1059.*(t664-t933).*(1.0./2.0);
t1285 = t659-t938+t1101+t1102;
t1286 = t89.*t668.*(1.0./2.0);
t1287 = t228.*t689.*(1.0./2.0);
t1288 = t32.*t854.*(1.0./2.0e2);
t1289 = t185+t1288;
t1294 = t31.*t854.*(3.0./1.0e3);
t1290 = t187-t1294;
t1292 = t25.*t313.*(1.6e1./5.0);
t1293 = -t698+t1106+t1107+t1292;
t1295 = t31.*t1290;
t1300 = t32.*t1289;
t1296 = t1295-t1300;
t1297 = t32.*t1290;
t1298 = t31.*t1289;
t1299 = t1297+t1298;
t1301 = t30.*t178.*t201.*(2.0./1.25e2);
t1306 = t30.*t202.*t854.*(2.0./1.25e2);
t1302 = t1301-t1306;
t1303 = t30.*t201.*t854.*(2.0./1.25e2);
t1304 = t30.*t178.*t202.*(2.0./1.25e2);
t1305 = t1303+t1304;
t1307 = t202.*t1302;
t1331 = t201.*t1305;
t1308 = t1307-t1331;
t1309 = t201.*t1302;
t1310 = t202.*t1305;
t1311 = t1309+t1310;
t1312 = t4.*t1311.*(1.0./2.0);
t1313 = -t248+t358+t359+t848;
t1314 = t1105.*t1313.*(1.0./2.0);
t1315 = t113+t224-t619-t1097;
t1316 = t1103.*t1315.*(1.0./2.0);
t1317 = t2.*t955.*(1.0./2.0);
t1318 = t4.*t1204.*(1.0./2.0);
t1319 = t124.*t1293.*(1.0./2.0);
t1320 = t1006.*t1105.*(1.0./2.0);
t1321 = t897.*t1293.*(1.0./2.0);
t1322 = t1285.*(t442-t937).*(1.0./2.0);
t1323 = t18.*t31.*(t949-t1234).*(1.0./2.0);
t1324 = t995.*t1103.*(1.0./2.0);
t1325 = t769.*t1204.*(1.0./2.0);
t1326 = t31.*t1207.*(3.0./5.0e2);
t1327 = t15.*t679.*(1.0./2.0);
t1328 = t15.*t686.*(1.0./2.0);
t1329 = t18.*t671.*(1.0./2.0);
t1330 = t18.*t675.*(1.0./2.0);
t1332 = t1094.*(t646-t903).*(1.0./2.0);
t1333 = t904.*(t1016-t1040).*(1.0./2.0);
t1334 = t30.*t62.*t854.*(1.1e1./1.0e3);
t1335 = t29.*t30.*t31.*t773.*(1.1e1./1.0e3);
t1356 = t30.*t330.*t854.*(1.0./2.0);
t1357 = t29.*t30.*t31.*t980.*(1.0./2.0);
t1336 = t1334+t1335-t1356-t1357;
t1337 = t840.*t1336.*(1.0./2.0);
t1338 = t30.*t178.*t773.*(1.1e1./1.0e3);
t1339 = t30.*t328.*t854.*(1.0./2.0);
t1340 = t30.*t178.*t980.*(1.0./2.0);
t1341 = t30.*t62.*t178.*(1.1e1./1.0e3);
t1342 = t29.*t30.*t31.*t328.*(1.0./2.0);
t1358 = t30.*t178.*t330.*(1.0./2.0);
t1359 = t29.*t30.*t31.*t43.*(1.1e1./1.0e3);
t1343 = t1341+t1342-t1358-t1359;
t1344 = t261.*t1177.*(1.0./2.0);
t1345 = t766.*(t384+t385-t693-t694).*(1.0./2.0);
t1346 = t1003.*t1048.*(1.0./2.0);
t1347 = t30.*t43.*t854.*(1.1e1./1.0e3);
t1348 = t1338+t1339+t1340+t1347;
t1349 = t835.*t1348.*(1.0./2.0);
t1350 = t901.*t1105.*(1.0./2.0);
t1351 = t897.*t1158.*(1.0./2.0);
t1352 = t486.*t689.*(1.0./2.0);
t1353 = t435.*t1148.*(1.0./2.0);
t1354 = t894.*(t680-t1151).*(1.0./2.0);
t1355 = t1150.*(t442-t937).*(1.0./2.0);
t1360 = t869.*t1270.*(1.0./2.0);
t1361 = t25.*t29.*t30.*t31.*(1.0./2.5e2);
t1362 = t15.*t1296.*(1.0./2.0);
t1363 = t18.*t955.*(1.0./2.0);
t1364 = t371.*t689.*(1.0./2.0);
t1365 = t110.*t1150.*(1.0./2.0);
t1367 = t15.*t940;
t1368 = t928+t1367;
t1369 = t25.*t940;
t1389 = t18.*t29.*t32.*(1.09e2./1.0e3);
t1370 = t1369-t1389;
t1371 = t32.*t771.*(3.0./1.0e3);
t1372 = t31.*t41.*(3.0./1.0e3);
t1373 = -t187+t1294+t1371+t1372;
t1374 = t32.*t41.*(1.0./2.0e2);
t1391 = t31.*t771.*(1.0./2.0e2);
t1375 = t185+t1288+t1374-t1391;
t1376 = t201.*t771.*(2.0./1.25e2);
t1377 = t41.*t202.*(2.0./1.25e2);
t1378 = t1376+t1377;
t1379 = t41.*t201.*(2.0./1.25e2);
t1394 = t202.*t771.*(2.0./1.25e2);
t1380 = t1379-t1394;
t1381 = t15.*t940.*(1.6e1./5.0);
t1382 = t18.*t506.*(1.6e1./5.0);
t1383 = t1381+t1382;
t1384 = t25.*t506.*(1.6e1./5.0);
t1385 = t15.*t29.*t32.*(2.18e2./6.25e2);
t1386 = t1384+t1385;
t1387 = t25.*t940.*(1.6e1./5.0);
t1406 = t18.*t29.*t32.*(2.18e2./6.25e2);
t1388 = t1387-t1406;
t1390 = t32.*t1373;
t1408 = t31.*t1375;
t1392 = t953+t954+t1390-t1408;
t1393 = t201.*t1378;
t1402 = t202.*t1380;
t1395 = t1393-t1402;
t1396 = t32.*t1375;
t1397 = t31.*t1373;
t1398 = t949-t1234+t1396+t1397;
t1399 = t201.*t1380;
t1400 = t202.*t1378;
t1401 = t1399+t1400;
t1403 = t110.*t1383.*(1.0./2.0);
t1404 = t87.*t931.*(1.0./2.0);
t1405 = t41.*t152.*(1.0./2.0);
t1407 = t124.*t1388.*(1.0./2.0);
t1409 = t2.*t1392.*(1.0./2.0);
t1410 = t2.*t1395.*(1.0./2.0);
t1411 = t4.*t1398.*(1.0./2.0);
t1412 = t4.*t1401.*(1.0./2.0);
t1413 = t178.*t1204.*(1.0./2.0);
t1414 = t854.*t955.*(1.0./2.0);
t1415 = t290.*t854.*(1.0./2.0);
t1416 = t29.*t32.*t62.*(1.0./2.5e2);
t1417 = t30.*t178.*t952.*(1.0./2.0);
t1418 = t30.*t854.*t947.*(1.0./2.0);
t1419 = t43.*t1401.*(1.0./2.0);
t1420 = t854.*t1308.*(1.0./2.0);
t1421 = t43.*t1311.*(1.0./2.0);
t1422 = t773.*t1308.*(1.0./2.0);
t1423 = t30.*t178.*t975.*(1.0./2.0);
t1424 = t30.*t817.*t854.*(1.0./2.0);
t1425 = t30.*t178.*(t317-t322).*(1.0./2.0);
t1477 = t517.*t634.*(1.0./2.0);
t1478 = t365.*t1117.*(1.0./2.0);
t1426 = t1228+t1229+t1230+t1231-t1477-t1478;
t1427 = t1032.*t1119.*(1.0./2.0);
t1428 = t869.*t1065.*(1.0./2.0);
t1429 = t169.*t952.*(1.0./2.0);
t1430 = t62.*(t545-t1070);
t1431 = t1069-t1255-t1256+t1430;
t1432 = t887.*t1032.*(1.0./2.0);
t1433 = t1240.*(t79-t826).*(1.0./2.0);
t1434 = t887.*(t1016-t1040).*(1.0./2.0);
t1435 = t992-t1077+t1081-t1085+t1086-t1087-t1088-t1091-t1092+t1257+t1258+t1259+t1332+t1333+t1345+t1425+t1433+t1434-t103.*t588.*(1.0./2.0)-t883.*t1015.*(1.0./2.0);
t1436 = t30.*t854.*(t42-t45).*(1.1e1./1.0e3);
t1437 = t1338+t1339+t1340+t1436;
t1438 = t169.*t201.*(2.0./1.25e2);
t1439 = t169.*t202.*(2.0./1.25e2);
t1446 = t201.*t827.*(2.0./1.25e2);
t1440 = t1439-t1446;
t1441 = t202.*t827.*(2.0./1.25e2);
t1442 = t1438+t1441;
t1443 = t43.*t1063.*(1.0./2.0);
t1444 = t328.*t827.*(1.0./2.0);
t1469 = t541.*t773.*(1.0./2.0);
t1470 = t169.*t980.*(1.0./2.0);
t1445 = t1443+t1444-t1469-t1470;
t1447 = t201.*t1440;
t1471 = t202.*t1442;
t1448 = t1447-t1471;
t1449 = t2.*t1448.*(1.0./2.0);
t1450 = t202.*t1440;
t1451 = t175.*t328.*(1.0./2.0);
t1452 = t169.*t330.*(1.0./2.0);
t1472 = t43.*t544.*(1.0./2.0);
t1473 = t62.*t541.*(1.0./2.0);
t1453 = t1451+t1452-t1472-t1473;
t1454 = t544.*t773.*(1.0./2.0);
t1455 = t62.*t1063.*(1.0./2.0);
t1474 = t175.*t980.*(1.0./2.0);
t1475 = t330.*t827.*(1.0./2.0);
t1456 = t1454+t1455-t1474-t1475;
t1457 = t218.*t1177.*(1.0./2.0);
t1458 = t107.*t1453.*(1.0./2.0);
t1459 = t1027.*t1058.*(1.0./2.0);
t1460 = t1022.*t1048.*(1.0./2.0);
t1461 = t201.*t1442;
t1462 = t1450+t1461;
t1463 = t4.*t1462.*(1.0./2.0);
t1464 = t1117.*(t104+t105).*(1.0./2.0);
t1465 = t1022.*(t646-t903).*(1.0./2.0);
t1466 = t1119.*(t81-t956).*(1.0./2.0);
t1467 = (t208+t1026).*(t664-t933).*(1.0./2.0);
t1468 = t1009+t1017+t1018-t1068-t1073-t1075;
t1476 = t15.*t31.*t975.*(1.0./2.0);
t1479 = t25.*t30.*(1.0./1.25e2);
t1480 = t29.*t32.*t33.*(1.0./1.25e2);
t1481 = t1479+t1480;
t1482 = t365.*t1453.*(1.0./2.0);
t1483 = t798.*t1445.*(1.0./2.0);
t1484 = t794.*t1456.*(1.0./2.0);
t1485 = t15.*t1311.*(1.0./2.0);
t1486 = t18.*t1308.*(1.0./2.0);
t1487 = t986+t991+t993+t994-t1228-t1229-t1230-t1231-t1241-t1361-t1476+t1477+t1478+t1485+t1486;
t1488 = t15.*t31.*(t973+t974).*(1.0./2.0);
t1489 = t517.*(t100+t101).*(1.0./2.0);
t1490 = t958.*(t395-t825).*(1.0./2.0);
t1491 = t960.*(t79-t826).*(1.0./2.0);
t1492 = (t204+t970).*(t431-t829).*(1.0./2.0);
t1494 = t202.*(t170-t828).*(2.0./1.25e2);
t1495 = t1438+t1494;
t1497 = t25.*t1481.*(1.0./2.0);
t1498 = t201.*t1495;
t1499 = t1450+t1498;
t1501 = t202.*t1495;
t1500 = t1447-t1501;
t1502 = t2.*t1500.*(1.0./2.0);
t1503 = t4.*t1499.*(1.0./2.0);
t1505 = t169.*t975.*(1.0./2.0);
t1506 = t43.*t1499.*(1.0./2.0);
t1507 = t175.*t821.*(1.0./2.0);
t1508 = t62.*t1481.*(1.0./2.0);
t1509 = t103.*t568.*(1.0./2.0);
t1510 = t321.*(t170-t828).*(1.0./2.0);
t1511 = t958.*t1032.*(1.0./2.0);
t1512 = t321.*t827.*(1.0./2.0);
t1513 = t958.*(t1016-t1040).*(1.0./2.0);
t1514 = t107.*t764.*(1.0./2.0);
t1515 = t62.*(t545-t1070).*(1.0./2.0);
t1516 = t1454-t1474-t1475+t1515;
t1517 = t840.*t989.*(1.0./2.0);
t1518 = t835.*t1055.*(1.0./2.0);
t1519 = t1048.*t1129.*(1.0./2.0);
t1520 = t1111+t1112+t1514+t1517+t1518+t1519-t356.*t1177.*(1.0./2.0)-t1058.*t1127.*(1.0./2.0);
t1521 = t792.*t1058.*(1.0./2.0);
t1522 = t365.*t764.*(1.0./2.0);
t1523 = t107.*t1219.*(1.0./2.0);
t1524 = t798.*t1055.*(1.0./2.0);
t1525 = t394.*t1177.*(1.0./2.0);
t1526 = t794.*t989.*(1.0./2.0);
t1527 = t1032.*t1055.*(1.0./2.0);
t1528 = t989.*t1015.*(1.0./2.0);
t1529 = t764.*t766.*(1.0./2.0);
t1530 = t1437.*(t81-t956).*(1.0./2.0);
t1531 = t1003.*(t1046-t1098).*(1.0./2.0);
t1538 = t840.*t1171.*(1.0./2.0);
t1540 = t838.*t1058.*(1.0./2.0);
t1532 = t1111+t1112+t1175+t1178+t1182+t1523-t1538-t1540;
t1533 = t968.*t1058.*(1.0./2.0);
t1534 = t960.*t1048.*(1.0./2.0);
t1535 = t517.*t1177.*(1.0./2.0);
t1536 = t15.*t1499.*(1.0./2.0);
t1537 = t15.*t965;
t1539 = t18.*t967.*(1.0./2.0);
t1541 = t29.*t821.*(1.0./2.0);
t1542 = t25.*t824.*(1.0./2.0);
t1543 = t365.*t1219.*(1.0./2.0);
t1544 = t794.*t1171.*(1.0./2.0);
t1545 = t794.*t1336.*(1.0./2.0);
t1546 = t365.*t1343.*(1.0./2.0);
t1547 = t889.*t1048.*(1.0./2.0);
t1548 = t494.*t1177.*(1.0./2.0);
t1549 = t798.*t1174.*(1.0./2.0);
t1550 = t1058.*t1209.*(1.0./2.0);
t1551 = t556.*t1177.*(1.0./2.0);
t1552 = t766.*t1219.*(1.0./2.0);
t1553 = t1048.*t1270.*(1.0./2.0);
t1554 = t1032.*t1174.*(1.0./2.0);
t1555 = t794.*t1516.*(1.0./2.0);
t1556 = t29.*t31.*t1481.*(1.0./2.0);
t1557 = t41.*t975;
t1558 = t771.*t817;
t1559 = t178.*t1311;
t1560 = t30.*t613.*t1205.*(1.0./1.25e2);
t1561 = t29.*t32.*t821;
t1562 = t986+t991+t993+t994+t1226-t1241-t1361-t1476+t1485+t1486-t1521+t1525-t1543-t1544-t1545-t1546-t1547+t1548+t1549+t1550-t798.*t1437.*(1.0./2.0);
t1563 = t999.*t1058.*(1.0./2.0);
t1564 = t107.*t1343.*(1.0./2.0);
t1565 = t2.*t1308.*(1.0./2.0);
t1566 = t1058.*t1080.*(1.0./2.0);
t1567 = t1015.*t1336.*(1.0./2.0);
t1568 = t1048.*t1240.*(1.0./2.0);
t1569 = t1032.*t1437.*(1.0./2.0);
t1573 = t29.*t30.*t31.*t62.*(1.0./2.5e2);
t1574 = t29.*t30.*t31.*t821.*(1.0./2.0);
t1582 = t588.*t1177.*(1.0./2.0);
t1583 = t766.*t1343.*(1.0./2.0);
t1570 = t1421+t1422+t1423+t1424+t1566+t1567+t1568+t1569-t1573-t1574-t1582-t1583;
t1571 = dq6.*t1570;
t1572 = t986+t991+t993+t994+t1226-t1241-t1312-t1337-t1344-t1488-t1521-t1522+t1524+t1525+t1526-t1530-t1531+t1563+t1564+t1565;
t1575 = t1009+t1017+t1018-t1068-t1073-t1075+t1482+t1483+t1497-t1533-t1534-t1535+t1536+t1555-t18.*t1500.*(1.0./2.0);
t1576 = t568.*t1177.*(1.0./2.0);
t1577 = t766.*t1453.*(1.0./2.0);
t1578 = t1048.*t1065.*(1.0./2.0);
t1579 = t1505+t1506+t1507+t1508+t1576+t1577+t1578-t817.*t827.*(1.0./2.0)-t773.*t1500.*(1.0./2.0)-t1032.*t1445.*(1.0./2.0)-t1058.*t1431.*(1.0./2.0)-t1015.*t1516.*(1.0./2.0);
t1580 = t1048.*t1094.*(1.0./2.0);
t1581 = t743.*t1177.*(1.0./2.0);
C = reshape([-dq4.*(t259+t262+t280+t287+t301+t307+t311+t528+t531-t2.*t284.*(1.0./2.0)-t2.*t290.*(1.0./2.0)-t4.*t289.*(1.0./2.0)-t155.*t181.*(1.0./2.0)-t161.*t178.*(1.0./2.0)-t94.*t299.*(1.0./2.0)-t98.*t296.*(1.0./2.0))+dq3.*(t372+t374+t377+t381+t383+t387+t402+t409+t471+t474+t110.*(t111+t112).*(1.0./2.0)+t116.*(t113+t117).*(1.0./2.0)-t18.*t152.*(1.0./2.0)-t15.*t161.*(1.0./2.0)-t2.*t406.*(1.0./2.0)-t4.*t411.*(1.0./2.0)+t165.*(t80+t275-t21.*t49-t36.*t53).*(1.0./2.0)+t83.*(t82+t370-t21.*t49.*(1.0./2.0)-t36.*t53.*(1.0./2.0)).*(1.0./2.0)+t121.*(t118-t10.*t29).*(1.0./2.0)+t124.*(t125-t10.*t29.*(1.6e1./5.0)).*(1.0./2.0))+dq2.*(t229+t233+t249+t251+t629+t235.*(t79-t36.*(t39+t30.*(t37+t32.*t35)).*(1.0./2.0)).*(1.0./2.0)+t110.*(t111+t112+t225-t4.*t7.*t15.*(8.0./5.0)).*(1.0./2.0)+t116.*(t113+t117+t224-t4.*t7.*t15.*(1.0./2.0)).*(1.0./2.0)+t4.*(t156+t158-t3.*t75-t7.*t78).*(1.0./2.0)-t2.*(t148+t149-t7.*t75-t3.*t146).*(1.0./2.0)-t94.*(t95+t243-t53.*t60-t49.*t65).*(1.0./2.0)-t103.*(t102+t239-t43.*t65-t51.*t60).*(1.0./2.0)-t98.*(t99+t245-t53.*t60.*(1.0./2.0)-t49.*t65.*(1.0./2.0)).*(1.0./2.0)-t107.*(t106+t241-t43.*t65.*(1.0./2.0)-t51.*t60.*(1.0./2.0)).*(1.0./2.0))-dq5.*t547-dq1.*t626,-dq2.*t626+dq6.*(t608+t612+t748+t1514-t83.*t739.*(1.0./2.0)-t356.*t742.*(1.0./2.0)-t357.*t751.*(1.0./2.0)+t98.*(t735+t736-t62.*t325.*(1.0./2.0)-t68.*t326.*(1.0./2.0)).*(1.0./2.0))-dq5.*(t197+t200+t206+t210+t219+t223-t608-t612)-dq4.*(t259+t262+t301+t307+t311-t512-t513-t514+t528+t531+t635+t638+t643+t645+t648+t672+t676+t682-t83.*(t439-t459+t640-t18.*t51.*(1.0./2.0)).*(1.0./2.0)-t155.*t181.*(1.0./2.0)-t161.*t178.*(1.0./2.0)-t4.*t679.*(1.0./2.0)-t4.*t686.*(1.0./2.0)-t89.*t668.*(1.0./2.0)-t110.*t661.*(1.0./2.0)-t228.*t689.*(1.0./2.0)-t360.*t657.*(1.0./2.0)-t124.*(t698+t699-t29.*t270.*(1.6e1./5.0)-t25.*t313.*(1.6e1./5.0)).*(1.0./2.0))-dq1.*(t229+t233+t249+t251+t627+t628+t629+t754+t2.*t152-t2.*t155-t4.*t161+t4.*t164+t2.*t342+t4.*t345+t4.*t347-t98.*t256.*(1.0./2.0)-t107.*t255.*(1.0./2.0)+t165.*t235.*(1.0./2.0)-t94.*t357.*(1.0./2.0)-t103.*t356.*(1.0./2.0)-t2.*t625-t2.*t631.*(1.0./2.0))+dq3.*(t372+t374+t461+t463+t471+t474-t635-t638-t639-t641-t643-t645-t648+t690+t700+t701+t702+t703+t706+t709+t710+t711+t724+t728+t2.*(t718-t31.*(t652+t31.*t35.*(1.0./2.0e2))).*(1.0./2.0)+t2.*(t714-t202.*(t649+t35.*t202.*(2.0./1.25e2))).*(1.0./2.0)),-dq2.*t1190-dq5.*(-t1111-t1112+t1122+t1123+t1124+t1125+t1126-t218.*t634.*(1.0./2.0))+dq6.*(t1111+t1112+t1175+t1178+t1181+t1182-t838.*t1058.*(1.0./2.0)-t840.*t1171.*(1.0./2.0))-dq4.*(t645+t672+t676-t1099-t1100+t1108+t1114+t1143+t1149+t1155+t1159+t1167+t1168+t1169+t1170+t1250-t178.*t411.*(1.0./2.0)-t261.*t634.*(1.0./2.0)-t371.*t689.*(1.0./2.0)-t2.*t1139.*(1.0./2.0)-t4.*t1140.*(1.0./2.0)-t110.*t1150.*(1.0./2.0)-t406.*t854.*(1.0./2.0)-t107.*t1154.*(1.0./2.0)-t634.*t705.*(1.0./2.0)-t838.*t1045.*(1.0./2.0)-t840.*t1044.*(1.0./2.0)-t999.*t1045.*(1.0./2.0))-dq3.*(t1109+t1110-t15.*t408.*(1.0./2.0)-t18.*t406.*(1.0./2.0))-dq1.*(t372+t374+t832+t836+t842+t843+t845+t847+t2.*t401-t2.*t406+t4.*t408-t4.*t411-t121.*t849.*(1.0./2.0)-t124.*t851.*(1.0./2.0)-t805.*t838.*(1.0./2.0)-t808.*t840.*(1.0./2.0)),dq1.*(t259+t262+t301-t512+t1004+t1005+t2.*t955+t4.*t1204-t2.*t1299-t840.*t883.*(1.0./2.0)-t805.*t999.*(1.0./2.0)-t4.*(t1295-t1300))+dq2.*(t259+t262+t301-t512+t635+t645+t672+t676+t1004+t1005-t1099-t1100+t1114-t1286-t1287+t1291+t1314+t1316+t1317+t1318+t1319-t4.*t1296.*(1.0./2.0)-t2.*t1299.*(1.0./2.0)-t110.*t1285.*(1.0./2.0)-t840.*t883.*(1.0./2.0)-t805.*t999.*(1.0./2.0)-t1127.*(t664-t933).*(1.0./2.0)-t840.*(t692+t793-t841-t934).*(1.0./2.0))-dq6.*(t1312+t1337+t1344+t1346+t1349-t2.*t1308.*(1.0./2.0)-t107.*t1343.*(1.0./2.0)-t999.*t1058.*(1.0./2.0))-dq5.*(t1122+t1123+t1124+t1125+t1126+t1312-t218.*t634.*(1.0./2.0)-t2.*t1308.*(1.0./2.0))+dq4.*(t1413+t1414-t178.*t1296.*(1.0./2.0)-t854.*t1299.*(1.0./2.0))+dq3.*(t645+t672+t676-t1099-t1100+t1114+t1143+t1149+t1155+t1159+t1167+t1168+t1169+t1170+t1362+t1363-t1154.*(t104+t105).*(1.0./2.0)-t371.*t689.*(1.0./2.0)-t2.*t1139.*(1.0./2.0)-t4.*t1140.*(1.0./2.0)-t110.*t1150.*(1.0./2.0)-t18.*t1299.*(1.0./2.0)-t261.*(t633-t662).*(1.0./2.0)-t705.*(t633-t662).*(1.0./2.0)-t15.*(t949-t1234).*(1.0./2.0)-t838.*(t664-t933).*(1.0./2.0)-t999.*(t664-t933).*(1.0./2.0)-t840.*(t692+t793-t841-t934).*(1.0./2.0)),dq4.*(t1122+t1312+t1464+t1465+t1466+t1467-t218.*t634.*(1.0./2.0)-t2.*t1308.*(1.0./2.0))-dq6.*(t1449+t1457+t1458+t1459+t1460+t1463-t835.*t1445.*(1.0./2.0)-t840.*t1456.*(1.0./2.0))+dq2.*(t219+t223+t1023+t1024+t1025+t1028-t1111-t1112)+dq3.*(-t1111-t1112+t1122+t1123+t1124+t1125+t1126-t218.*(t633-t662).*(1.0./2.0))+dq1.*(t219+t223+t1023+t1024+t1025+t1028),dq5.*(t1457+t1458+t1459+t1460+t1502+t1503-t840.*t1516.*(1.0./2.0)-(t81-t956).*(t1443+t1444-t1469-t1470).*(1.0./2.0))-dq2.*t1520-dq3.*t1532+dq4.*(t1312+t1337+t1344+t1530+t1531-t2.*t1308.*(1.0./2.0)-t107.*t1343.*(1.0./2.0)-t999.*t1058.*(1.0./2.0)),dq3.*(t366+t369+t372+t374+t377+t381+t383+t387+t390+t393+t397+t402+t409+t461+t463+t465+t466+t472+t473+t475+t476+t165.*(t80+t275-t354-t21.*t49).*(1.0./2.0)-t2.*t406.*(1.0./2.0)-t4.*t411.*(1.0./2.0)+t83.*t425.*(1.0./2.0)-t21.*(t317-t322).*(1.0./2.0))+dq1.*(t229+t233+t249+t251+t627+t628+t752+t753-t98.*t256.*(1.0./2.0)-t107.*t255.*(1.0./2.0)-t94.*t357.*(1.0./2.0)-t103.*t356.*(1.0./2.0)+t4.*(t156+t362-t3.*t75-t7.*t78).*(1.0./2.0)-t2.*(t148+t149-t246-t247).*(1.0./2.0))-dq5.*(t197+t200+t206+t210+t219+t223+t323-t53.*t321.*(1.0./2.0))+dq2.*(t343+t344+t346+t348+t349-t255.*(t104+t105)-t356.*(t100+t101)-t2.*t155.*(1.0./2.0)-t4.*t161.*(1.0./2.0)+t87.*t228+t83.*t237+t89.*t232-t98.*t256+t124.*t254+t110.*t272+t165.*t235-t94.*t357+t116.*t351+t121.*t360-t2.*t625.*(1.0./2.0)-t2.*t631+t4.*t632)+dq4.*(-t259-t262-t280-t287-t301-t307-t311+t366+t369+t390+t393+t397+t452+t453+t454+t512+t513+t514+t394.*(t100+t101).*(1.0./2.0)+t2.*t284.*(1.0./2.0)+t4.*t289.*(1.0./2.0)-t232.*t435.*(1.0./2.0)-t254.*(t445+t25.*(t8+t9-t2.*t32.*(1.09e2./1.0e3)+t31.*t35.*(1.09e2./1.0e3))).*(1.0./2.0)-t87.*(t436+t530-t25.*t268-t29.*t266).*(1.0./2.0)-t116.*(t440+t526-t35.*t266-t15.*t313).*(1.0./2.0)-t121.*(t451+t533-t29.*t270-t25.*t313).*(1.0./2.0)+t272.*(t442-t15.*t270).*(1.0./2.0)-t15.*t31.*t318.*(1.0./2.0))-dq6.*(t323+t597-t53.*t321.*(1.0./2.0)-t256.*t422.*(1.0./2.0)-t255.*t427.*(1.0./2.0)+t94.*(t428+t592-t62.*t325-t68.*t326).*(1.0./2.0)+t103.*(t419+t596-t62.*t333-t68.*t328).*(1.0./2.0)-t165.*(t415+t593-t51.*t326-t49.*t333).*(1.0./2.0)),dq2.*(t229+t233+t627+t628+t752+t753+t754+(t3.*t755.*(3.3e1./2.5e2)+t3.*t756.*(3.3e1./2.5e2)).*(t7.*t755.*(2.97e2./6.25e2)+t7.*t756.*(2.97e2./6.25e2)).*(1.0./2.0)+(t7.*t755.*(3.3e1./2.5e2)+t7.*t756.*(3.3e1./2.5e2)).*(t3.*t755.*(2.97e2./6.25e2)+t3.*t756.*(2.97e2./6.25e2)).*(1.0./2.0)-t98.*t256.*(1.0./2.0)-t107.*t255.*(1.0./2.0)-t94.*t357.*(1.0./2.0)-t103.*t356.*(1.0./2.0)-t2.*t631.*(1.0./2.0)+t124.*(t125+t250-t252-t253).*(1.0./2.0)+t121.*(t118+t248-t358-t359).*(1.0./2.0)-t3.*t7.*t755.*6.27264e-2-t3.*t7.*t756.*6.27264e-2)-dq1.*t626+dq3.*(t369+t372+t374+t393+t461+t463+t472+t488+t499-t635-t638-t643-t645-t648+t663+t690+t696+t700+t701+t702+t703+t706+t709+t710+t711+t724+t728-t21.*t318.*(1.0./2.0)+t164.*(t22-t38).*(1.0./2.0)+t321.*(t22-t38).*(1.0./2.0)+t2.*(t718-t31.*t720).*(1.0./2.0)+t2.*(t714-t202.*t716).*(1.0./2.0))+dq6.*(-t323-t597+t608-t734-t744+t748+t1095+t764.*(t104+t105).*(1.0./2.0)+t256.*t422.*(1.0./2.0)+t4.*t763.*(1.0./2.0)-t83.*t739.*(1.0./2.0)-t356.*t742.*(1.0./2.0)-t357.*t751.*(1.0./2.0)+(t79-t194).*(t415+t593-t594-t49.*t333).*(1.0./2.0)+t321.*(t52-t69).*(1.0./2.0)+t98.*(t735+t736-t62.*(-t22+t38+t56+t324-t412).*(1.0./2.0)-t68.*t326.*(1.0./2.0)).*(1.0./2.0))-dq5.*(t197+t200+t206+t210+t219+t223+t323-t535-t608-t612)+dq4.*(-t259-t262-t301-t307-t311+t369+t393+t452+t453+t454+t488+t499+t512+t513+t514-t635-t638-t643-t645-t648+t663-t672-t676-t682+t683+t690+t696+t1099+t1100+t1286+t1287-t232.*t435.*(1.0./2.0)-t87.*t665.*(1.0./2.0)-t254.*t498.*(1.0./2.0)+t110.*t661.*(1.0./2.0)-t116.*t658.*(1.0./2.0)-t121.*t697.*(1.0./2.0)+t124.*(t698+t699-t29.*t270.*(1.6e1./5.0)-t25.*t313.*(1.6e1./5.0)).*(1.0./2.0)+t657.*(t118+t248-t358-t359).*(1.0./2.0)-t15.*t31.*t318.*(1.0./2.0)),-dq5.*(-t1033-t1038-t1043-t1111-t1112+t1122+t1123+t1124+t1125+t1126+t1172+t1183+t1184-t218.*t634.*(1.0./2.0))+dq3.*(t870-t880-t881+t1130+t1131+t1132+t1133+t1134+t1135+t1136+t1160-t18.*t874.*(1.0./2.0)-t25.*t919.*(1.0./2.0)-t25.*t924.*(1.0./2.0)-t29.*t921.*(1.0./2.0)-t29.*t926.*(1.0./2.0)-(t664-t933).*(t448+t791-t806-t852).*(1.0./2.0)-(t431-t829).*(t692+t793-t841-t934).*(1.0./2.0))-dq1.*t1190-dq4.*(t645+t672+t676-t870+t880+t881-t1099-t1100+t1114+t1138+t1143+t1149+t1155-t1156+t1159-t1160+t1161+t1162+t1163+t1164+t1165+t1166+t1167+t1168+t1169+t1170+t1212+t1213-t261.*t634.*(1.0./2.0)-t371.*t689.*(1.0./2.0)-t2.*t1139.*(1.0./2.0)-t4.*t1140.*(1.0./2.0)-t110.*t1150.*(1.0./2.0)-t107.*t1154.*(1.0./2.0)-t634.*t705.*(1.0./2.0)-t854.*t877.*(1.0./2.0)-t838.*t1045.*(1.0./2.0)-t999.*t1045.*(1.0./2.0)-t15.*t31.*t401.*(1.0./2.0)-t15.*t31.*t914.*(1.0./2.0)-t25.*t31.*t921.*(1.0./2.0)-t25.*t31.*t926.*(1.0./2.0))+dq6.*(t1033+t1038+t1111+t1112-t1172+t1175+t1178+t1181+t1182-t1183-t1184+t1195+t1220+t1279+t1284-t644.*t766.*(1.0./2.0)-t838.*t1058.*(1.0./2.0)-t904.*t1032.*(1.0./2.0)-t869.*t1094.*(1.0./2.0)-t840.*t1171.*(1.0./2.0))-dq2.*(t372+t374+t706+t709+t832+t836+t845+t847-t107.*t644+t2.*t874-t2.*t877+t4.*t907+t4.*t910-t121.*t849.*(1.0./2.0)-t124.*t851.*(1.0./2.0)-t356.*t634-t805.*t838.*(1.0./2.0)-t808.*t840.*(1.0./2.0)-t835.*t904+t840.*t1044-t869.*t1129+t1045.*t1127),-dq5.*(-t1087-t1088-t1092+t1122+t1123+t1124+t1125+t1126+t1257+t1258+t1259+t1312-t218.*t634.*(1.0./2.0)-t2.*t1308.*(1.0./2.0))-dq4.*(-t870+t880+t881-t1160+t1232+t1233+t1235+t1236+t1251+t1252+t1320+t1321+t1322+t1323+t1324-t435.*t668.*(1.0./2.0)-t665.*t689.*(1.0./2.0)-t671.*t854.*(1.0./2.0)-t675.*t854.*(1.0./2.0)-t25.*t29.*t613.*(3.0./2.5e2)-t18.*t31.*t947.*(1.0./2.0))+dq1.*(t259+t262+t301-t512+t635+t645+t672+t676+t1004+t1005-t1099-t1100+t1114-t1286-t1287+t1291+t1314+t1316+t1317+t1318+t1319-t2.*t1299.*(1.0./2.0)-t110.*t1285.*(1.0./2.0)-t840.*t883.*(1.0./2.0)-t805.*t999.*(1.0./2.0)-t4.*(t1295-t1300).*(1.0./2.0)-t1127.*(t664-t933).*(1.0./2.0)-t840.*(t692+t793-t841-t934).*(1.0./2.0))+dq3.*(t645+t672+t676+t870-t880-t881-t1099-t1100+t1114+t1143+t1149+t1155+t1159+t1160+t1167+t1168+t1169+t1170-t1201-t1202-t1203-t1206-t1251-t1252+t1325+t1326+t1327+t1328+t1329+t1330-t1154.*(t104+t105).*(1.0./2.0)-t371.*t689.*(1.0./2.0)-t2.*t1139.*(1.0./2.0)-t4.*t1140.*(1.0./2.0)-t110.*t1150.*(1.0./2.0)-t261.*(t633-t662).*(1.0./2.0)-t705.*(t633-t662).*(1.0./2.0)-t838.*(t664-t933).*(1.0./2.0)-t999.*(t664-t933).*(1.0./2.0)-t840.*(t692+t793-t841-t934).*(1.0./2.0))-dq6.*(-t1077-t1085-t1087-t1088-t1091-t1092+t1257+t1258+t1259+t1312+t1332+t1333+t1337+t1344+t1345+t1346+t1349-t2.*t1308.*(1.0./2.0)-t107.*t1343.*(1.0./2.0)-t999.*t1058.*(1.0./2.0))+dq2.*(t259+t262+t301-t512+t1004+t1005+t2.*t671+t2.*t675-t4.*t679-t4.*t686+t107.*t644-t89.*t668-t228.*t689+t356.*t634-t110.*t1285+t124.*t1293-t840.*t883.*(1.0./2.0)+t835.*t904-t805.*t999.*(1.0./2.0)+t869.*t1129+t1103.*t1315+t1105.*t1313-t1127.*(t664-t933)-t840.*(t692+t793-t841-t934)),-dq5.*t1468-dq6.*(t1009+t1017+t1018-t1068-t1073-t1075+t1449+t1457+t1458+t1459+t1460+t1463-t835.*t1445.*(1.0./2.0)-t840.*t1456.*(1.0./2.0))+dq2.*(t219+t223+t1023+t1024+t1025+t1028-t2.*t967-t4.*t965)+dq1.*(t219+t223+t1023+t1024+t1025+t1028-t1111-t1112)+dq4.*(-t986-t991-t993-t994+t1122+t1241+t1312+t1464+t1465+t1466+t1467+t1488-t218.*t634.*(1.0./2.0)-t2.*t1308.*(1.0./2.0))+dq3.*(t818-t1111-t1112+t1122+t1123+t1124+t1125+t1126+t1196+t1199-t25.*t824.*(1.0./2.0)-t29.*t821.*(1.0./2.0)-t18.*t967.*(1.0./2.0)-t218.*(t633-t662).*(1.0./2.0)),-dq1.*t1520-dq4.*t1572-dq2.*(t107.*t764+t2.*t967+t4.*t965-t356.*t1177+t840.*t989+t835.*t1055+t1048.*t1129-t1058.*t1127)+dq6.*(-t1009-t1017-t1018+t1068+t1073+t1075+t1527+t1528+t1529+t1580+t1581-t1058.*t1059.*(1.0./2.0))-dq3.*(-t818+t1111+t1112+t1175+t1178+t1182-t1196-t1199+t1226-t1521-t1522+t1523+t1524+t1525+t1526+t1539+t1541+t1542-t838.*t1058.*(1.0./2.0)-t840.*t1171.*(1.0./2.0))+dq5.*(-t1009-t1017-t1018+t1068+t1073+t1075+t1457+t1458+t1459+t1460+t1502+t1503-t840.*t1516.*(1.0./2.0)-(t81-t956).*(t1443+t1444-t1469-t1470).*(1.0./2.0)),-dq6.*(t323+t554+t555+t557+t559-t53.*t321.*(1.0./2.0)-t165.*t551.*(1.0./2.0)+t424.*t425.*(1.0./2.0))+dq5.*(t515+t520+t523+t535-t517.*(t100+t101).*(1.0./2.0)-t94.*t522.*(1.0./2.0)-t51.*(t317-t322).*(1.0./2.0)-t199.*(t395-t432).*(1.0./2.0))+dq2.*(t366+t369+t372+t374+t377+t381+t383+t387+t393+t397+t461+t463+t465+t466+t469+t470-t471+t472+t473-t474+t475+t476+t639+t641+t165.*t458.*(1.0./2.0)-t21.*(t317-t322).*(1.0./2.0))+dq3.*(t790+t795+t1109+t1110-t21.*t318-t15.*t408.*(1.0./2.0)-t18.*t406.*(1.0./2.0)+t94.*t392-t368.*t380-t365.*t386+t164.*(t22-t38)+t321.*(t22-t38)+t458.*(t79-t194)+t460.*(t395-t432))+dq1.*(t372+t374+t377+t381+t383+t387+t461+t463+t465+t466+t469+t470)+dq4.*(t393+t452+t453+t454+t477+t480+t487+t488+t489+t491+t495+t496+t499+t503-t18.*t279.*(1.0./2.0)+t15.*t286.*(1.0./2.0)+t18.*t284.*(1.0./2.0)-t15.*t289.*(1.0./2.0)-t94.*t479.*(1.0./2.0)-t116.*t490.*(1.0./2.0)-t165.*t483.*(1.0./2.0)-t296.*t368.*(1.0./2.0)-t310.*t396.*(1.0./2.0)-t368.*t380.*(1.0./2.0)-t365.*t386.*(1.0./2.0)-t373.*t435.*(1.0./2.0)-t446.*t498.*(1.0./2.0)-t15.*t31.*t318.*(1.0./2.0)),dq4.*(t452+t453+t454+t477+t480+t487+t495+t496+t499-t866-t870+t878+t879+t880+t881+t884+t885+t890+t891+t895+t898+t902+t1201+t1202+t1203+t1206-t18.*t671.*(1.0./2.0)-t18.*t675.*(1.0./2.0)-t15.*t679.*(1.0./2.0)-t15.*t686.*(1.0./2.0)-t373.*t435.*(1.0./2.0)-t116.*t894.*(1.0./2.0)-t365.*t708.*(1.0./2.0)-t31.*t1207.*(3.0./5.0e2)-t794.*t808.*(1.0./2.0)-t798.*t887.*(1.0./2.0)-t801.*t889.*(1.0./2.0)-t798.*t904.*(1.0./2.0)-t769.*t1204.*(1.0./2.0)-t15.*t31.*t318.*(1.0./2.0))+dq1.*(t372+t374+t471-t472+t474-t499-t639-t641-t663+t832+t836+t842+t843+t845+t847+t866+t1007+t1191+t1192+t1193-t121.*t849.*(1.0./2.0)-t124.*t851.*(1.0./2.0)-t805.*t838.*(1.0./2.0)-t808.*t840.*(1.0./2.0)-t797.*(t79-t826).*(1.0./2.0)-t1001.*(t395-t825).*(1.0./2.0))-dq5.*(t323-t515+t818+t819+t957+t959+t961+t969+t972+t1196+t1199-t25.*t824.*(1.0./2.0)-t29.*t821.*(1.0./2.0)-t18.*t967.*(1.0./2.0))-dq6.*(t323+t555+t557+t559+t767+t818+t819+t1039+t1522+t21.*(t202.*(t768-t49.*t201.*(2.0./1.25e2))+t201.*(t770+t49.*t202.*(2.0./1.25e2))).*(1.0./2.0)-t165.*t551.*(1.0./2.0)+t15.*t763.*(1.0./2.0)-t25.*t824.*(1.0./2.0)-t29.*t821.*(1.0./2.0)+t396.*t739.*(1.0./2.0)-t394.*t742.*(1.0./2.0)-t392.*t751.*(1.0./2.0)-t458.*t777.*(1.0./2.0)-t794.*t989.*(1.0./2.0)-t18.*(t606-t202.*t761).*(1.0./2.0))-dq3.*(-t790-t795+t870+t1130+t1131+t1132+t1133+t1134+t1135+t1136+t21.*t318-t18.*t874.*(1.0./2.0)+t164.*t769-t25.*t919.*(1.0./2.0)-t25.*t924.*(1.0./2.0)-t29.*t921.*(1.0./2.0)-t29.*t926.*(1.0./2.0)-t365.*t644.*(1.0./2.0)-t394.*t634.*(1.0./2.0)+t365.*t708+t321.*t769+t792.*t805-t797.*t801-t798.*t803+t794.*t808-t794.*(t692+t793-t25.*t776.*(1.0./2.0)-t29.*t773.*(1.0./2.0)).*(1.0./2.0)+t798.*(t712+t871-t21.*t773.*(1.0./2.0)-t43.*t769.*(1.0./2.0)).*(1.0./2.0)-t792.*(t664-t25.*t773.*(1.0./2.0)).*(1.0./2.0))+dq2.*(t372+t374+t832+t836+t842+t843+t845+t847-t121.*t849.*(1.0./2.0)-t124.*t851.*(1.0./2.0)-t805.*t838.*(1.0./2.0)-t808.*t840.*(1.0./2.0)),-dq1.*(t472+t499-t645-t866+t890+t891+t1109+t1110-t1114+t1156-t1168+t1186+t1187+t1188-t1191-t1192-t1193-t1194+t1210+t1211-t15.*t408.*(1.0./2.0)-t18.*t406.*(1.0./2.0)-t365.*t708.*(1.0./2.0)-t794.*t808.*(1.0./2.0))-dq2.*(t472+t499-t645-t866-t870+t880+t881+t890+t891-t1114-t1130-t1131-t1132-t1133-t1134-t1135-t1136+t1156-t1160-t1168+t1186+t1187+t1188-t1191-t1192-t1193-t1194+t1210+t1211+t1212+t1213+t1214+t1215+t1216+t1217+t1218-t365.*t708.*(1.0./2.0)-t794.*t808.*(1.0./2.0))-dq6.*(t818-t1033-t1038+t1172+t1183+t1184-t1195+t1196+t1199-t1220-t1226+t1264+t1272+t1521+t1543+t1544-t25.*t824.*(1.0./2.0)-t29.*t821.*(1.0./2.0)-t18.*t967.*(1.0./2.0)-t556.*t634.*(1.0./2.0)-t394.*t1177.*(1.0./2.0)-t798.*t1174.*(1.0./2.0)+t869.*t1224.*(1.0./2.0)-t1045.*t1227.*(1.0./2.0))-dq5.*(t818-t1033-t1038+t1172+t1183+t1184-t1195+t1196+t1199+t1228+t1229+t1230+t1231-t25.*t824.*(1.0./2.0)-t29.*t821.*(1.0./2.0)-t18.*t967.*(1.0./2.0)-t517.*t634.*(1.0./2.0)-t365.*t1117.*(1.0./2.0))-dq4.*(t1138+t1161+t1162+t1163+t1164+t1165+t1166-t1201-t1202-t1203-t1206+t1244+t1245+t1246+t1247+t1248+t1249+t1325+t1326+t1327+t1328+t1329+t1330-t18.*t1139.*(1.0./2.0)-t854.*t877.*(1.0./2.0)-t1045.*t1209.*(1.0./2.0)-t15.*t31.*t401.*(1.0./2.0)-t15.*t31.*t914.*(1.0./2.0)-t25.*t31.*t921.*(1.0./2.0)-t25.*t31.*t926.*(1.0./2.0))+dq3.*(t870-t880-t881+t1130+t1131+t1132+t1133+t1134+t1135+t1136+t1160-t1214-t1215-t1216-t1217-t1218-(t664-t933).*(t448+t791-t806-t852).*(1.0./2.0)-(t431-t829).*(t692+t793-t841-t934).*(1.0./2.0)),-dq1.*(t477+t480+t495+t496-t645-t672-t676+t884+t885+t1099+t1100-t1114-t1149-t1155+t1156-t1159-t1168-t1170+t1210+t1211-t1362-t1363+t1364+t1365+t15.*t1204.*(1.0./2.0)+t18.*t1299.*(1.0./2.0)-t798.*t887.*(1.0./2.0)-t801.*t889.*(1.0./2.0))-dq2.*(t477+t480+t495+t496-t645-t672-t676-t870+t880+t881+t884+t885+t1099+t1100-t1114-t1149-t1155+t1156-t1159-t1160-t1168-t1170+t1201+t1202+t1203+t1206+t1210+t1211+t1251+t1252-t1325-t1326-t1327-t1328-t1329-t1330+t1364+t1365-t798.*t887.*(1.0./2.0)-t801.*t889.*(1.0./2.0))-dq5.*(-t1087-t1088-t1092+t1228+t1229+t1230+t1231+t1257+t1258+t1259+t1361-t517.*t634.*(1.0./2.0)-t15.*t1311.*(1.0./2.0)-t18.*t1308.*(1.0./2.0)-t365.*t1117.*(1.0./2.0))-dq4.*(-t870+t880+t881-t1160+t1232+t1233+t1235+t1236+t1251+t1252+t1323+t1350+t1351+t1352+t1353+t1354+t1355-t671.*t854.*(1.0./2.0)-t675.*t854.*(1.0./2.0)-t25.*t29.*t613.*(3.0./2.5e2)-t18.*t31.*t947.*(1.0./2.0))-dq6.*(-t1087-t1088-t1092-t1220+t1257+t1258+t1259+t1264+t1272+t1360+t1361+t1545+t1546+t1547-t556.*t634.*(1.0./2.0)-t15.*t1311.*(1.0./2.0)-t18.*t1308.*(1.0./2.0)-t494.*t1177.*(1.0./2.0)+t798.*t1348.*(1.0./2.0)-t1058.*t1209.*(1.0./2.0)-t1045.*t1227.*(1.0./2.0))+dq3.*(t1244+t1245+t1246+t1247+t1248+t1249+t18.*t671+t18.*t675+t15.*t679+t15.*t686-t21.*t952-t21.*t955-t18.*t1139.*(1.0./2.0)-t31.*t1205.*(3.0./2.5e2)+t31.*t1207.*(3.0./2.5e2)+t797.*t869+t798.*t904-t769.*t947+t769.*t1204-(t507-t935).*(t664-t933).*(1.0./2.0)-(t633-t662).*(t292+t293-t449-t450)-(t364-t444).*(t384+t385-t693-t694)-(t664-t933).*(t448+t791-t806-t852)-(t431-t829).*(t692+t793-t841-t934)),-dq5.*t1468-dq4.*t1487+dq6.*(-t1009-t1017-t1018+t1068+t1073+t1075+t1482+t1483+t1484+t1497-t18.*t1448.*(1.0./2.0)+t15.*t1462.*(1.0./2.0)-t517.*t1177.*(1.0./2.0)-t968.*t1058.*(1.0./2.0)-t960.*(t1046-t1098).*(1.0./2.0))+dq1.*(t957+t959+t961+t969+t972-t1111-t1112-t222.*(t364-t444).*(1.0./2.0))+dq2.*(t818+t957+t959+t961+t969+t972-t1111-t1112+t1196+t1199-t25.*t824.*(1.0./2.0)-t29.*t821.*(1.0./2.0)-t18.*t967.*(1.0./2.0)-t222.*(t364-t444).*(1.0./2.0))+dq3.*(t1228+t1229+t1230+t1231+t1537-t25.*t824-t29.*t821-t18.*t967+t21.*t975+t769.*t817-t517.*(t633-t662).*(1.0./2.0)-t1117.*(t364-t444).*(1.0./2.0)),-dq1.*t1532-dq4.*t1562-dq5.*t1575+dq6.*(-t1009-t1017-t1018+t1068+t1073+t1075+t1551+t1552+t1553+t1554-t1015.*(t1060+t1061-t1221-t1222).*(1.0./2.0)-t1058.*(t1041+t1042-t1261-t1262).*(1.0./2.0))+dq3.*(t1537+t21.*(t973+t974)-t25.*t824-t29.*t821-t18.*t967-t394.*t1177-t797.*t1048-t798.*t1174+(t364-t444).*(t746-t985+t1179+t1180)+t1058.*(t448+t791-t806-t852)+t769.*(t816-t202.*(t770+t812))+(t431-t829).*(t1060+t1061-t1221-t1222))-dq2.*(-t818+t1111+t1112+t1175+t1178+t1182-t1196-t1199+t1226-t1521-t1522+t1523+t1524+t1525+t1526-t1538+t1539-t1540+t1541+t1542),dq3.*(t393+t452+t453+t454+t477+t480+t487+t488+t489+t491+t495+t496+t499+t503+t1108-t94.*t479.*(1.0./2.0)+t181.*t401.*(1.0./2.0)-t181.*t406.*(1.0./2.0)-t178.*t411.*(1.0./2.0)-t116.*t490.*(1.0./2.0)-t165.*t483.*(1.0./2.0)-t296.*t368.*(1.0./2.0)-t310.*t396.*(1.0./2.0)-t368.*t380.*(1.0./2.0)-t365.*t386.*(1.0./2.0)-t373.*t435.*(1.0./2.0)-t446.*t498.*(1.0./2.0)-t15.*t31.*t318.*(1.0./2.0))+dq6.*(t524+t525+t579+t585+t589+t590-t588.*(t100+t101).*(1.0./2.0)-t296.*t422.*(1.0./2.0))+dq5.*(t515+t520+t523+t524+t525-t517.*(t100+t101).*(1.0./2.0)-t94.*t522.*(1.0./2.0)-t199.*(t395-t432).*(1.0./2.0))-dq4.*(t939+t944+t121.*(t25.*t510-t18.*t29.*t32.*(1.09e2./1.0e3))-t41.*t152+t47.*t164+t47.*t321+t181.*t279.*(1.0./2.0)+t178.*t286.*(1.0./2.0)-t181.*t284.*(1.0./2.0)-t178.*t289.*(1.0./2.0)-t181.*t290+t94.*t479-t103.*t494-t258.*t365+t165.*t483+t296.*t368+t310.*t396-t87.*t931+t116.*(t928+t15.*t510))+dq2.*(-t259-t262-t301-t307-t311+t369+t393+t452+t453+t454+t488+t499+t512+t513+t514+t528+t531+t663+t683+t696-t155.*t181.*(1.0./2.0)-t161.*t178.*(1.0./2.0)-t232.*t435.*(1.0./2.0)-t87.*t665.*(1.0./2.0)-t254.*t498.*(1.0./2.0)-t116.*t658.*(1.0./2.0)-t121.*t697.*(1.0./2.0)-t15.*t31.*t318.*(1.0./2.0))-dq1.*(t259+t262+t301+t307+t311-t512-t513-t514),dq6.*(t524+t986+t991+t992+t993+t994+t1081+t1086+t1226+t1432+t1524+t1526-t588.*(t100+t101).*(1.0./2.0)+t394.*t742.*(1.0./2.0)-t883.*t1015.*(1.0./2.0)+t801.*(t1082+t1083+t1084+t30.*t43.*t854.*(1.1e1./5.0e2)).*(1.0./2.0)-t1058.*(t448+t791-t806-t852).*(1.0./2.0)-(t364-t444).*(t745+t746-t984-t985).*(1.0./2.0)-t15.*t31.*(t973+t974).*(1.0./2.0)-t25.*t31.*t821.*(1.0./2.0))-dq1.*(t259+t262+t301+t366+t452+t453+t454+t476-t512+t528-t866+t1004+t1005-t1007-t161.*t178.*(1.0./2.0)-t232.*t435.*(1.0./2.0)-t87.*t665.*(1.0./2.0)+t152.*t854.*(1.0./2.0)-t155.*t854.*(1.0./2.0)-t116.*t995.*(1.0./2.0)+t121.*t1006.*(1.0./2.0)+t797.*t801.*(1.0./2.0)-t840.*t883.*(1.0./2.0)+t798.*t1001.*(1.0./2.0)-t805.*t999.*(1.0./2.0)+t897.*(-t250+t252+t253+t850).*(1.0./2.0)+t997.*(t111+t225-t352-t863).*(1.0./2.0)-t15.*t31.*t318.*(1.0./2.0))+dq4.*(-t870+t878+t879+t880+t881-t939-t944+t1232+t1233+t1235+t1236+t1320+t1321+t1322+t1324+t494.*(t100+t101)+t41.*t152-t164.*t771+t87.*t931-t321.*t771-t435.*t668.*(1.0./2.0)+t290.*t854-t665.*t689.*(1.0./2.0)-t116.*t1368-t121.*t1370-t671.*t854.*(1.0./2.0)-t675.*t854.*(1.0./2.0)-t798.*t887-t801.*t889-t798.*t904.*(1.0./2.0)+t258.*(t364-t444)+t883.*(t431-t829)+t805.*(t507-t935)-t25.*t29.*t613.*(3.0./2.5e2)-t18.*t31.*t947.*(1.0./2.0)+t18.*t31.*t1204.*(1.0./2.0))-dq2.*(t259+t262+t301-t512+t1004+t1005-t840.*t883.*(1.0./2.0)-t805.*t999.*(1.0./2.0))+dq5.*(t515+t524-t957-t959-t961-t969-t972+t986+t991+t992+t993+t994-t25.*t31.*t821.*(1.0./2.0)-t15.*t31.*t975.*(1.0./2.0))+dq3.*(t452+t453+t454+t477+t480+t487+t495+t496+t499-t866-t870+t878+t879+t880+t881+t884+t885+t890+t891+t895+t898+t902+t1138+t1161+t1162+t1163+t1164+t1165+t1166-t373.*t435.*(1.0./2.0)-t116.*t894.*(1.0./2.0)-t365.*t708.*(1.0./2.0)-t794.*t808.*(1.0./2.0)-t798.*t887.*(1.0./2.0)-t801.*t889.*(1.0./2.0)-t798.*t904.*(1.0./2.0)-t854.*t877.*(1.0./2.0)-t15.*t31.*t318.*(1.0./2.0)-t15.*t31.*t401.*(1.0./2.0)-t15.*t31.*t914.*(1.0./2.0)-t25.*t31.*t921.*(1.0./2.0)-t25.*t31.*t926.*(1.0./2.0)),-dq3.*(t1244+t1245+t1246+t1247+t1248+t1249-t18.*t1139.*(1.0./2.0)-t1045.*t1209.*(1.0./2.0))-dq1.*(t452+t453+t454+t487+t499-t866+t890+t891+t895+t898+t902+t1108+t1143+t1167+t1169+t1250-t178.*t411.*(1.0./2.0)-t373.*t435.*(1.0./2.0)-t261.*t634.*(1.0./2.0)-t116.*t894.*(1.0./2.0)-t365.*t708.*(1.0./2.0)-t2.*t1139.*(1.0./2.0)-t4.*t1140.*(1.0./2.0)-t406.*t854.*(1.0./2.0)-t107.*t1154.*(1.0./2.0)-t794.*t808.*(1.0./2.0)-t999.*t1045.*(1.0./2.0)-t15.*t31.*t318.*(1.0./2.0))+dq6.*(t986+t991+t993+t994+t1226-t1241-t1242-t1243+t1260+t1265+t1266+t1267+t1268+t1271+t1525+t1549-t766.*t1154.*(1.0./2.0)-(t364-t444).*(t746-t985+t1179+t1180).*(1.0./2.0)-t1058.*(t448+t791-t806-t852).*(1.0./2.0)-(t431-t829).*(t1060+t1061-t1221-t1222).*(1.0./2.0)-t15.*t31.*(t973+t974).*(1.0./2.0))-dq5.*(-t986-t991-t993-t994+t1228+t1229+t1230+t1231+t1241+t1242+t1243+t1476-t517.*t634.*(1.0./2.0)-t365.*t1117.*(1.0./2.0)-t29.*t30.*t31.*t921.*(1.0./2.0))+dq4.*(-t870+t880+t881-t1160+t1232+t1233+t1235+t1236+t1251+t1252+t1323+t1350+t1351+t1352+t1353+t1354+t1355+t41.*t401+t41.*t914-t494.*t634+t411.*t771+t178.*t1140-t365.*t1154-t671.*t854.*(1.0./2.0)-t675.*t854.*(1.0./2.0)+t771.*t916-t869.*t889-t794.*t1142-t798.*t1146+t854.*t1139+(t507-t935).*(t664-t933)-t25.*t29.*t613.*(3.0./2.5e2)+t29.*t32.*t921+t29.*t32.*t926-t18.*t31.*t947.*(1.0./2.0))-dq2.*(t452+t453+t454+t487+t499-t866-t870+t880+t881+t890+t891+t895+t898+t902+t1138+t1143-t1160+t1161+t1162+t1163+t1164+t1165+t1166+t1167+t1169+t1251+t1252-t373.*t435.*(1.0./2.0)-t261.*t634.*(1.0./2.0)-t116.*t894.*(1.0./2.0)-t365.*t708.*(1.0./2.0)-t2.*t1139.*(1.0./2.0)-t4.*t1140.*(1.0./2.0)-t107.*t1154.*(1.0./2.0)-t794.*t808.*(1.0./2.0)-t854.*t877.*(1.0./2.0)-t999.*t1045.*(1.0./2.0)-t15.*t31.*t318.*(1.0./2.0)-t15.*t31.*t401.*(1.0./2.0)-t15.*t31.*t914.*(1.0./2.0)-t25.*t31.*t921.*(1.0./2.0)-t25.*t31.*t926.*(1.0./2.0)),-dq4.*(t1244+t1245+t1247+t1248+t1249+t41.*t952.*(1.0./2.0)+t41.*t955.*(1.0./2.0)+t178.*t1398.*(1.0./2.0)+t178.*t1401.*(1.0./2.0)+t689.*t931.*(1.0./2.0)+t771.*t947.*(1.0./2.0)+t435.*t1386.*(1.0./2.0)-t771.*t1204.*(1.0./2.0)+t854.*t1392.*(1.0./2.0)+t854.*t1395.*(1.0./2.0)-t1045.*t1209.*(1.0./2.0)-t897.*t1388.*(1.0./2.0)+t997.*t1383.*(1.0./2.0)+t1103.*t1368.*(1.0./2.0)-t1105.*t1370.*(1.0./2.0)-t31.*t32.*t1205.*(3.0./2.5e2))-dq5.*(t1228+t1229+t1230+t1231-t1416-t1417-t1418-t1419-t1420+t41.*t975.*(1.0./2.0)-t517.*t634.*(1.0./2.0)-t365.*t1117.*(1.0./2.0)+t178.*t1311.*(1.0./2.0)+t771.*t817.*(1.0./2.0)+t773.*t1395.*(1.0./2.0)+t29.*t32.*t821.*(1.0./2.0))-dq3.*(-t870+t880+t881-t1160+t1232+t1233+t1235+t1236+t1251+t1252+t1323+t1350+t1351+t1352+t1353+t1354+t1355+t41.*t401.*(1.0./2.0)+t41.*t914.*(1.0./2.0)+t411.*t771.*(1.0./2.0)+t178.*t1140.*(1.0./2.0)+t18.*t1392.*(1.0./2.0)-t15.*t1398.*(1.0./2.0)+t18.*t1395.*(1.0./2.0)-t15.*t1401.*(1.0./2.0)-t671.*t854.*(1.0./2.0)-t675.*t854.*(1.0./2.0)+t771.*t916.*(1.0./2.0)+t854.*t1139.*(1.0./2.0)-t25.*t29.*t32.*(3.0./5.0e2)-t25.*t29.*t613.*(3.0./2.5e2)+t29.*t32.*t921.*(1.0./2.0)+t29.*t32.*t926.*(1.0./2.0)-t18.*t31.*t947.*(1.0./2.0))-dq2.*(t495+t496-t870+t880+t881+t884+t885+t1143-t1160+t1167+t1169+t1232+t1233+t1235+t1236+t1251+t1252+t1320+t1321+t1322+t1323+t1324+t1403+t1404+t1405+t1407+t1409+t1410+t1411+t1412+t1415-t41.*t318.*(1.0./2.0)-t178.*t300.*(1.0./2.0)-t261.*t634.*(1.0./2.0)-t164.*t771.*(1.0./2.0)-t321.*t771.*(1.0./2.0)-t435.*t668.*(1.0./2.0)-t107.*t1154.*(1.0./2.0)-t665.*t689.*(1.0./2.0)-t89.*t1386.*(1.0./2.0)-t116.*t1368.*(1.0./2.0)-t121.*t1370.*(1.0./2.0)-t671.*t854.*(1.0./2.0)-t675.*t854.*(1.0./2.0)-t798.*t887.*(1.0./2.0)-t801.*t889.*(1.0./2.0)-t999.*t1045.*(1.0./2.0)-t25.*t29.*t613.*(3.0./2.5e2)-t18.*t31.*t947.*(1.0./2.0))+dq6.*(t1265+t1266+t1267+t1268+t1271+t1416+t1417+t1418+t1419+t1420+t1548+t1550-t41.*(t973+t974).*(1.0./2.0)-t178.*t1311.*(1.0./2.0)-t766.*t1154.*(1.0./2.0)-t773.*t1395.*(1.0./2.0)-t1343.*(t364-t444).*(1.0./2.0)-t1336.*(t431-t829).*(1.0./2.0)-t1437.*(t395-t825).*(1.0./2.0)-t889.*(t1046-t1098).*(1.0./2.0)-t771.*(t816-t202.*(t770+t812)).*(1.0./2.0)-t29.*t32.*t821.*(1.0./2.0))-dq1.*(t495+t496+t884+t885+t1143+t1167+t1169+t1403+t1404+t1405+t1407+t1409+t1410+t1411+t1412-t1413-t1414+t1415-t41.*t318.*(1.0./2.0)-t178.*t300.*(1.0./2.0)-t261.*t634.*(1.0./2.0)-t164.*t771.*(1.0./2.0)-t321.*t771.*(1.0./2.0)-t107.*t1154.*(1.0./2.0)+t178.*t1296.*(1.0./2.0)-t89.*t1386.*(1.0./2.0)-t116.*t1368.*(1.0./2.0)-t121.*t1370.*(1.0./2.0)-t798.*t887.*(1.0./2.0)-t801.*t889.*(1.0./2.0)-t999.*t1045.*(1.0./2.0)+t854.*t1299.*(1.0./2.0)),dq2.*(-t515+t969-t986-t991-t993-t994+t1241+t1312+t1488+t1489+t1490+t1491+t1492-t2.*t1308.*(1.0./2.0))-dq3.*t1487-dq5.*(t1421+t1422+t1423+t1424-t29.*t30.*t31.*t62.*(1.0./2.5e2)-t29.*t30.*t31.*t821.*(1.0./2.0))-dq6.*(t1421+t1422+t1423+t1424-t1482-t1483-t1484+t1533+t1534+t1535+t178.*t1462.*(1.0./2.0)+t854.*t1448.*(1.0./2.0)-t29.*t31.*t1481.*(1.0./2.0)-t29.*t30.*t31.*t62.*(1.0./2.5e2)-t29.*t30.*t31.*t821.*(1.0./2.0))+dq4.*(t1228+t1229+t1230+t1231+t1557+t1558+t1559+t1560+t1561-t517.*(t633-t662).*(1.0./2.0)-t1117.*(t364-t444).*(1.0./2.0)-t854.*(t1307-t1331))+dq1.*(-t515+t969+t1312+t1489+t1490+t1491+t1492-t2.*t1308.*(1.0./2.0)),-t1571-dq5.*(t1421+t1422+t1423+t1424+t1482+t1483-t1533-t1534-t1535+t1555+t1556-t178.*t1499.*(1.0./2.0)-t854.*t1500.*(1.0./2.0)-t29.*t30.*t31.*t62.*(1.0./2.5e2)-t29.*t30.*t31.*t821.*(1.0./2.0))-dq3.*t1562-dq2.*t1572+dq4.*(t1557+t1558+t1559+t1560+t1561-t494.*t1177+t365.*t1343+t889.*t1048+t794.*t1336+t798.*t1437-t1058.*(t507-t935)-t854.*(t1307-t1331))+dq1.*(t1312+t1337+t1344+t1530+t1531-t1563-t1564-t1565),-dq2.*(t197+t200+t206+t210+t219+t223+t323-t535)-dq1.*t547+dq4.*(t515+t520+t523+t524+t525-t517.*(t100+t101).*(1.0./2.0)-t94.*t522.*(1.0./2.0)-t199.*(t395-t432).*(1.0./2.0))+dq3.*(t515+t520+t523+t535-t517.*(t100+t101).*(1.0./2.0)-t94.*t522.*(1.0./2.0)-t51.*(t317-t322).*(1.0./2.0)-t199.*(t395-t432).*(1.0./2.0))+dq6.*(t564+t565+t572+t573+t574+t575+t1012-t321.*(t170-t172).*(1.0./2.0))+dq5.*(t169.*t318-t321.*(t170-t172)),dq5.*(t1009+t1017+t1018-t43.*t965.*(1.0./2.0)-t51.*t975.*(1.0./2.0)-t321.*t827-t776.*t817.*(1.0./2.0)+t169.*(t317-t322))-dq3.*(t323-t515+t819+t957+t959+t961+t969+t972+t1033+t1038+t1043-t62.*t919.*(1.0./2.0)-t68.*t921.*(1.0./2.0)-t773.*t874.*(1.0./2.0))-dq1.*(t219+t223-t323-t819+t1023+t1024+t1025+t1028)-dq4.*(-t515-t524+t957+t959+t961+t969+t972-t992+t1087+t1088+t1092-t51.*t952.*(1.0./2.0)-t776.*t947.*(1.0./2.0)-t29.*t31.*t68.*(1.0./2.5e2))+dq6.*(t1009+t1012+t1017+t1018+t1066+t1067+t1074+t1076+t1511-t43.*t965.*(1.0./2.0)-t51.*t975.*(1.0./2.0)-t321.*t827.*(1.0./2.0)-t776.*t817.*(1.0./2.0)-t805.*t1072.*(1.0./2.0))-dq2.*(t219+t223+t1023+t1024+t1025+t1028),-dq4.*(t1087+t1088+t1092+t1228+t1229+t1230+t1231+t1242+t1243-t1257-t1258-t1259-t1260-t517.*t634.*(1.0./2.0)-t365.*t1117.*(1.0./2.0))-dq2.*(-t323-t819-t1033-t1038-t1043+t1122+t1123+t1124+t1125+t1126+t1172+t1183+t1184-t218.*t634.*(1.0./2.0))+dq6.*t1278-dq3.*t1426-dq1.*(-t323-t819+t1122+t1123+t1124+t1125+t1126-t218.*t634.*(1.0./2.0))-dq5.*(-t1009-t1017-t1018+t1068+t1073+t1075+t169.*t914+t175.*t921-t827.*t916),-dq4.*t1426-dq2.*(t992-t1087-t1088-t1092+t1122+t1123+t1124+t1125+t1126+t1257+t1258+t1259+t1425-t218.*t634.*(1.0./2.0))-dq3.*(-t1087-t1088-t1092+t1228+t1229+t1230+t1231-t1242-t1243+t1257+t1258+t1259+t1260-t517.*t634.*(1.0./2.0)-t365.*t1117.*(1.0./2.0))-dq1.*(t992+t1122+t1123+t1124+t1125+t1126+t1425-t218.*t634.*(1.0./2.0))+dq6.*(t1274+t1276+t1421+t1422+t1423+t1424+t1427+t1428+t1429-t568.*(t633-t662).*(1.0./2.0)-t947.*(t170-t828).*(1.0./2.0)-t1431.*(t664-t933).*(1.0./2.0)-t29.*t31.*t175.*(1.0./2.5e2)-t29.*t30.*t31.*t62.*(1.0./2.5e2)-t29.*t30.*t31.*t821.*(1.0./2.0))+dq5.*(t1421+t1422+t1423+t1424+t169.*t952-t947.*(t170-t828)-t29.*t31.*t175.*(1.0./1.25e2)-t29.*t30.*t31.*t62.*(1.0./2.5e2)-t29.*t30.*t31.*t821.*(1.0./2.0)),dq2.*(-t1009-t1017-t1018-t1067+t1068+t1073+t1075+t1502+t1503+t1512)-dq3.*(t1009+t1017+t1018-t1068-t1073-t1075+t1273-t1493-t1496+t1497+t1536-t18.*t1500.*(1.0./2.0))+dq1.*(-t565+t1502+t1503+t1510)-dq5.*(t1505+t1506+t1507+t1508-t817.*t827.*(1.0./2.0)-t773.*t1500.*(1.0./2.0))-dq4.*(t1421+t1422+t1423+t1424+t1429+t1556-t178.*t1499.*(1.0./2.0)-t827.*t947.*(1.0./2.0)-t854.*t1500.*(1.0./2.0)-t29.*t31.*t175.*(1.0./2.5e2)-t29.*t30.*t31.*t62.*(1.0./2.5e2)-t29.*t30.*t31.*t821.*(1.0./2.0)),dq1.*(t1457+t1458+t1459+t1460+t1502+t1503-t840.*t1516.*(1.0./2.0)-(t81-t956).*(t1443+t1444-t1469-t1470).*(1.0./2.0))-dq3.*t1575-dq6.*t1579-dq4.*(t1421+t1422+t1423+t1424+t1482+t1483-t1533-t1534-t1535+t1555+t1556-t1573-t1574-t178.*t1499.*(1.0./2.0)-t854.*t1500.*(1.0./2.0))-dq5.*(t175.*t821+t169.*t975+t43.*t1499+t62.*t1481-t817.*t827-t773.*t1500)+dq2.*(-t1009-t1017-t1018+t1068+t1073+t1075+t1457+t1458+t1459+t1460+t1502+t1503-t840.*t1516.*(1.0./2.0)-(t81-t956).*(t1443+t1444-t1469-t1470).*(1.0./2.0)),dq4.*(t524+t525+t579+t585+t589+t590-t588.*(t100+t101).*(1.0./2.0)-t296.*t422.*(1.0./2.0))-dq2.*(t323-t535+t597+t734+t744-t165.*(t415+t593-t594-t49.*t333).*(1.0./2.0)-t256.*t422.*(1.0./2.0)-t255.*t427.*(1.0./2.0))+dq5.*(t564+t565+t572+t573+t574+t575+t1509-t321.*(t170-t172).*(1.0./2.0))-dq3.*(t323-t535+t554+t555+t557+t559+t767-t165.*t551.*(1.0./2.0)),-dq6.*(-t1009-t1017-t1018+t1068+t1073+t1075+t1527+t1528+t1529+t742.*t743.*(1.0./2.0)+t1048.*t1050.*(1.0./2.0)-t1058.*t1059.*(1.0./2.0))+dq4.*t1435+dq5.*(t1009+t1012+t1017+t1018+t1066+t1067-t1068-t1073+t1074-t1075+t1076+t1513-t321.*t827.*(1.0./2.0)-t805.*t1072.*(1.0./2.0))+dq1.*(t323+t744+t819-t1095-t805.*t1059.*(1.0./2.0)+t801.*t1094.*(1.0./2.0)-t996.*t1015.*(1.0./2.0)+t1001.*t1032.*(1.0./2.0))-dq3.*(t323+t557+t819+t1033+t1038+t1039+t1043+t1077+t1085+t1091-t62.*t919.*(1.0./2.0)-t68.*t921.*(1.0./2.0)-t644.*t766.*(1.0./2.0)-t773.*t874.*(1.0./2.0)-t808.*t1015.*(1.0./2.0)+t803.*t1032.*(1.0./2.0)-t869.*t1050.*(1.0./2.0)-t904.*t1032.*(1.0./2.0)+t801.*t1224.*(1.0./2.0)-t805.*t1227.*(1.0./2.0)),dq5.*t1278-dq6.*(-t1009-t1017-t1018+t1068+t1073+t1075+t1551+t1552+t1553+t1554-t1015.*t1171.*(1.0./2.0)-t1058.*t1227.*(1.0./2.0))+dq1.*(t819+t1039+t1280+t1281+t1282+t1283-t808.*t1015.*(1.0./2.0)-t805.*t1227.*(1.0./2.0))+dq2.*(t819+t1033+t1038+t1039-t1172-t1183-t1184+t1195+t1220-t1264-t1272+t1279+t1280+t1281+t1282+t1283+t1284-t808.*t1015.*(1.0./2.0)-t869.*t1094.*(1.0./2.0)-t805.*t1227.*(1.0./2.0))+dq4.*(-t1092-t1220-t1242-t1243+t1257+t1258+t1259+t1260+t1264+t1265+t1266+t1267+t1268+t1271+t1272+t1360-t766.*t1154.*(1.0./2.0)-t686.*(t42-t45).*(1.0./2.0)-t773.*(t674-t868).*(1.0./2.0)-(t633-t662).*(t419+t552+t553-t595).*(1.0./2.0)-(t664-t933).*(t1041+t1042-t1261-t1262).*(1.0./2.0)),t1571-dq2.*t1435-dq1.*(t524+t992+t1081+t1086+t1432-t103.*t588.*(1.0./2.0)-t883.*t1015.*(1.0./2.0)+t801.*t1240.*(1.0./2.0))-dq3.*(-t1087-t1088-t1092-t1220-t1242-t1243+t1257+t1258+t1259+t1260+t1264+t1265+t1266+t1267+t1268+t1271+t1272+t1360-t556.*t634.*(1.0./2.0)-t766.*t1154.*(1.0./2.0)-t1045.*t1227.*(1.0./2.0))+dq5.*(t1274+t1276+t1421+t1422+t1423+t1424+t1427+t1428+t1429-t568.*(t633-t662).*(1.0./2.0)-t947.*(t170-t828).*(1.0./2.0)-t1431.*(t664-t933).*(1.0./2.0)-t29.*t31.*t175.*(1.0./2.5e2)-t29.*t30.*t31.*t62.*(1.0./2.5e2)-t29.*t30.*t31.*t821.*(1.0./2.0)),dq6.*(t1505+t1506+t1507+t1508+t1576+t1577+t1578-t773.*t1500.*(1.0./2.0)-t1058.*t1431.*(1.0./2.0)-t1015.*t1516.*(1.0./2.0)-(t1016-t1040).*(t1443+t1444-t1469-t1470).*(1.0./2.0)-(t170-t828).*(t816-t202.*(t770+t812)).*(1.0./2.0))-dq1.*(t565+t1076+t1509-t1510+t1511+t801.*t1065.*(1.0./2.0)+t971.*t1015.*(1.0./2.0)-t805.*t1431.*(1.0./2.0))-dq4.*(t1274+t1276+t1421+t1422+t1423+t1424+t1427+t1428+t1429-t1504-t827.*t947.*(1.0./2.0)-t1045.*t1431.*(1.0./2.0)-t29.*t31.*t175.*(1.0./2.5e2)-t29.*t30.*t31.*t62.*(1.0./2.5e2)-t29.*t30.*t31.*t821.*(1.0./2.0))-dq2.*(t1009+t1012+t1017+t1018+t1066+t1067-t1068-t1073+t1074-t1075+t1076-t1512+t1513-t805.*t1431.*(1.0./2.0))-dq3.*(t1009+t1017+t1018-t1068-t1073-t1075+t1273+t1274+t1275+t1276+t1277-t1493-t1496-t1504-t1045.*t1431.*(1.0./2.0)),-dq4.*t1570-dq5.*t1579+dq3.*(-t1009-t1017-t1018+t1068+t1073+t1075+t1551+t1552+t1553+t1554-t1015.*(t1060+t1061-t1221-t1222).*(1.0./2.0)-t1058.*(t1041+t1042-t1261-t1262).*(1.0./2.0))+dq2.*(-t1009-t1017-t1018+t1068+t1073+t1075+t1527+t1528+t1529+t1580+t1581-t1058.*t1059.*(1.0./2.0))],[6,6]);
